simulink subsystem "PvtSubSys_VSM_ALL"  (R2020b)
settings: Solver=VariableStepAuto  StartTime=0.0  StopTime=10.0  RelTol=1e-3
values from neighbouring files (symbols this model uses):
  P_VSM_NOH_Act_Req = 0    [VSM_All.sldd]
  P_VSM_NOH_Swt_Req = 0    [VSM_All.sldd]
undefined symbols (not defined in the file or in its folder): ACC_STATE, HWA_STATE, LCK_STATE, P_VSM_ACCSOS_SW, P_VSM_AESSwtReq, P_VSM_CruiseFunUserInputMappingWays, P_VSM_ELKSwtReq, P_VSM_ESS_VehSwtReq, P_VSM_HWA_DMS_Enable, P_VSM_ICA_HandsOffSwtReq, P_VSM_IntelligentEvaSwtReq, P_VSM_ISLSwtReq, P_VSM_LCKSwtReq, P_VSM_LDWSwtReq, P_VSM_LKASwtReq, P_VSM_LSSSwtReq, P_VSM_PowerTrainConfig, P_VSM_SOSContinueTime, P_VSM_SOSSpdLimit, P_VSM_TSR_Dis_keep_SPL_Table, P_VSM_TSR_Dis_keep_SPLend, P_VSM_TSR_Dis_keep_TS_Table, P_VSM_TSR_Ena_SPLSupp_Table, P_VSM_TSR_Ena_TS_Table, P_VSM_TSR_SLIF_Speed_High, P_VSM_TSR_SLIF_Speed_Low, P_VSM_TSR_SLW_SnvtySwitch, P_VSM_TSR_SLW_Speed_Delta_disable, P_VSM_TSR_SLW_Speed_Delta_enable, P_VSM_TSR_SLW_Speed_High, P_VSM_TSR_SLW_Speed_Low, P_VSM_TSR_SLW_TrafEyeAvtiveDist, P_VSM_TSR_SLW_Warning_Time, P_VSM_TSR_SteerWheelAngle, P_VSM_TSR_SWS_speed_withDir, P_VSM_TSR_SWS_speed_woDir, P_VSM_TSRSwtReq, P_VSM_TSRWarnSwtReq, TJA_STATE, User_LC_ALCswt, User_LC_DrvConfirm, User_LC_DrvLCswt, User_LC_DrvOverride, User_LC_LeTurnNextLineReq, User_LC_RiTurnNextLineReq, User_LC_TurnMostLeLineReq, User_LC_TurnMostRiLineReq, User_LeTurnLmpOn, User_RiTurnLmpOn
libraries: simulink x51
(part 2 of 7)

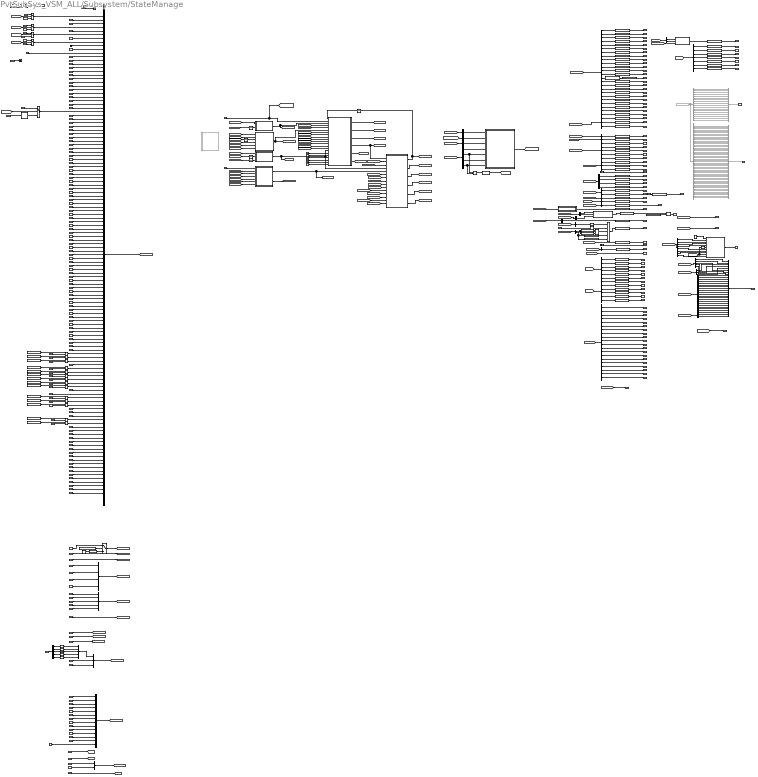
== system PvtSubSys_VSM_ALL/Subsystem/StateManage ==
  note: GotoFrom颜色说明
      | 前景色-背景色
      | Black-Orange 模块输入(连接到本模块输入端口)
      | Black-Cyan 模块输出(仅连接到本模块输出端口)
      | Blue-Cyan 模块输出(连接到本模块输出端口同时被其他模块使用)
      | Blue-others 内部跳转(未连接到本模块输入输入端口)
      | Black-White 未指定/其他
  note: 0:ICE
      | 1:PHEV
  note: 版本管理
      | VSM
      | 20201203-4.0
      | 初版
  note: 换道点灯信号
  note: 配置自
  note: 诊断
  note: 脱手检测
  EngState_PHEV : Inport  OutDataTypeStr=uint8  PortDimensions=1
  EngSpd : Inport  Port=2  OutDataTypeStr=single  PortDimensions=1
  EngState : Inport  Port=3
  BrkPedalSts : Inport  Port=4
  Start_StopSts : Inport  Port=5
  AccPedalOverride : Inport  Port=6
  AccelPedlPosnDiagc : Inport  Port=7
  ECMRespACC : Inport  Port=8
  ECMACCInterface : Inport  Port=9
  AccelPedalPosn : Inport  Port=10
  EngLimpHomeSts : Inport  Port=11
  CurrentGearValid : Inport  Port=12  OutDataTypeStr=boolean  PortDimensions=1
  SHIFT_IN_PROGRESS : Inport  Port=13  OutDataTypeStr=boolean  PortDimensions=1
  TargetGearValid : Inport  Port=14  OutDataTypeStr=boolean  PortDimensions=1
  TARGET_GEAR : Inport  Port=15  OutDataTypeStr=uint8  PortDimensions=1
  ShiftInPrgValid : Inport  Port=16  OutDataTypeStr=boolean  PortDimensions=1
  CURRENT_GEAR : Inport  Port=17  OutDataTypeStr=uint8  PortDimensions=1
  TGS_LEVER : Inport  Port=18  OutDataTypeStr=uint8  PortDimensions=1
  HCU_BrkPedalSts : Inport  Port=19  OutDataTypeStr=uint8  PortDimensions=1
  HCU_AccelPedalPosn_Diag : Inport  Port=20  OutDataTypeStr=single  PortDimensions=1
  HCU_ACCInterface : Inport  Port=21  OutDataTypeStr=boolean  PortDimensions=1
  HCU_PowertrainSts : Inport  Port=22  OutDataTypeStr=uint8  PortDimensions=1
  ACU_ShiftInProgress : Inport  Port=23  OutDataTypeStr=boolean  PortDimensions=1
  HCU_DrvMod : Inport  Port=24  OutDataTypeStr=uint8  PortDimensions=1
  HCU_PTDrvMod : Inport  Port=25  OutDataTypeStr=uint8  PortDimensions=1
  DrvTrqReqOvld : Inport  Port=26  OutDataTypeStr=boolean  PortDimensions=1
  HCU_GearSts : Inport  Port=27  OutDataTypeStr=uint8  PortDimensions=1
  DrivingModDis : Inport  Port=28
  BrkDskOvrheatd : Inport  Port=29  OutDataTypeStr=boolean  PortDimensions=1
  NoBrkForce : Inport  Port=30  OutDataTypeStr=boolean  PortDimensions=1
  VehStandstill : Inport  Port=31  OutDataTypeStr=uint8  PortDimensions=1
  HDCCtrl : Inport  Port=32  OutDataTypeStr=uint8  PortDimensions=1
  CDDActv : Inport  Port=33  OutDataTypeStr=boolean  PortDimensions=1
  CDDAvailable : Inport  Port=34  OutDataTypeStr=boolean  PortDimensions=1
  AVHSts : Inport  Port=35  OutDataTypeStr=uint8  PortDimensions=1
  ESPFuncOffSts : Inport  Port=36  OutDataTypeStr=boolean  PortDimensions=1
  ESPBrkLmpCtrl : Inport  Port=37  OutDataTypeStr=boolean  PortDimensions=1
  ESPFailSts : Inport  Port=38  OutDataTypeStr=boolean  PortDimensions=1
  ESP_MasterCylBrkPressVld : Inport  Port=39  OutDataTypeStr=boolean  PortDimensions=1
  MSRActv : Inport  Port=40  OutDataTypeStr=boolean  PortDimensions=1
  VDCActv : Inport  Port=41  OutDataTypeStr=boolean  PortDimensions=1
  PTCActv : Inport  Port=42  OutDataTypeStr=boolean  PortDimensions=1
  BTCActv : Inport  Port=43  OutDataTypeStr=boolean  PortDimensions=1
  ESP_MasterCylBrkPress : Inport  Port=44  OutDataTypeStr=single  PortDimensions=1
  MSRActv_RA : Inport  Port=45  OutDataTypeStr=boolean  PortDimensions=1
  PTCActv_RA : Inport  Port=46  OutDataTypeStr=boolean  PortDimensions=1
  BTCActv_RA : Inport  Port=47  OutDataTypeStr=boolean  PortDimensions=1
  ABSFailSts : Inport  Port=48  OutDataTypeStr=boolean  PortDimensions=1
  EBDFailSts : Inport  Port=49  OutDataTypeStr=boolean  PortDimensions=1
  VehSpd : Inport  Port=50  OutDataTypeStr=single  PortDimensions=1
  ABSActv : Inport  Port=51  OutDataTypeStr=boolean  PortDimensions=1
  EPBSts : Inport  Port=52  OutDataTypeStr=uint8  PortDimensions=1
  EPB_SwtPosn : Inport  Port=53  OutDataTypeStr=uint8  PortDimensions=1
  RLWheelDriveDirection : Inport  Port=54  OutDataTypeStr=uint8  PortDimensions=1
  RLWheelSpd : Inport  Port=55  OutDataTypeStr=single  PortDimensions=1
  RRWheelDriveDirection : Inport  Port=56  OutDataTypeStr=uint8  PortDimensions=1
  RRWheelSpd : Inport  Port=57  OutDataTypeStr=single  PortDimensions=1
  EPS_FailSts : Inport  Port=58  OutDataTypeStr=uint8  PortDimensions=1
  EPS_TrqSnsrSts : Inport  Port=59  OutDataTypeStr=boolean  PortDimensions=1
  EPS_SteerMod : Inport  Port=60  OutDataTypeStr=uint8  PortDimensions=1
  EPS_LKATorqOvrlDlvd : Inport  Port=61  OutDataTypeStr=single  PortDimensions=1
  EPS_LKATorqOvrlDlvdVld : Inport  Port=62  OutDataTypeStr=boolean  PortDimensions=1
  EPS_LKATrqOvlDlvdSts : Inport  Port=63  OutDataTypeStr=uint8  PortDimensions=1
  EPS_DrvInpTrqVal_HighReslolution : Inport  Port=64  OutDataTypeStr=single  PortDimensions=1
  SysPowerMod : Inport  Port=65  OutDataTypeStr=uint8  PortDimensions=1
  WiprReq : Inport  Port=66  OutDataTypeStr=uint8  PortDimensions=1
  DrvDoorSts : Inport  Port=67  OutDataTypeStr=boolean  PortDimensions=1
  PassengerDoorSts : Inport  Port=68  OutDataTypeStr=boolean  PortDimensions=1
  WindshldWiprActvSts : Inport  Port=69  OutDataTypeStr=boolean  PortDimensions=1
  HazardLmpSwtSts : Inport  Port=70  OutDataTypeStr=boolean  PortDimensions=1
  "KL30BRelaySts " : Inport  Port=71  OutDataTypeStr=boolean  PortDimensions=1
  ACAmbTemp : Inport  Port=72  OutDataTypeStr=single  PortDimensions=1
  HoodSts_F_Pbox : Inport  Port=73  OutDataTypeStr=boolean  PortDimensions=1
  FFogLmpSts_F_Pbox : Inport  Port=74  OutDataTypeStr=boolean  PortDimensions=1
  RFogLmpSts_R_Pbox : Inport  Port=75  OutDataTypeStr=boolean  PortDimensions=1
  LowBeamSts : Inport  Port=76  OutDataTypeStr=boolean  PortDimensions=1
  FrntWshrSwtSts : Inport  Port=77  OutDataTypeStr=uint8  PortDimensions=1
  FrntWiprSwtSts : Inport  Port=78  OutDataTypeStr=uint8  PortDimensions=1
  LTurnLmpSwtSts : Inport  Port=79  OutDataTypeStr=boolean  PortDimensions=1
  RTurnLmpSwtSts : Inport  Port=80  OutDataTypeStr=boolean  PortDimensions=1
  SteerWheelAng : Inport  Port=81  OutDataTypeStr=single  PortDimensions=1
  SteerWheelAngSign : Inport  Port=82  OutDataTypeStr=boolean  PortDimensions=1
  SteerWheelSpd : Inport  Port=83  OutDataTypeStr=single  PortDimensions=1
  SteerWheelSpdSign : Inport  Port=84  OutDataTypeStr=boolean  PortDimensions=1
  SAS_Sts : Inport  Port=85  OutDataTypeStr=uint8  PortDimensions=1
  ACC_TimeGap_IncSetSwt : Inport  Port=86  OutDataTypeStr=boolean  PortDimensions=1
  ACC_TimeGap_DecSetSwt : Inport  Port=87  OutDataTypeStr=boolean  PortDimensions=1
  CC_ACC_CRUISE_OFFSwt : Inport  Port=88  OutDataTypeStr=boolean  PortDimensions=1
  CC_ACC_CANCEL_OFFSwt : Inport  Port=89  OutDataTypeStr=boolean  PortDimensions=1
  CC_ACC_IncSetSpd_ResuSwt : Inport  Port=90  OutDataTypeStr=boolean  PortDimensions=1
  CC_ACC_DecSetSpd_SetSwt : Inport  Port=91  OutDataTypeStr=boolean  PortDimensions=1
  CC_ACCSwtErr : Inport  Port=92  OutDataTypeStr=boolean  PortDimensions=1
  HWA_OK_OFFSwt : Inport  Port=93  OutDataTypeStr=boolean  PortDimensions=1
  DrvSBR : Inport  Port=94  OutDataTypeStr=boolean  PortDimensions=1
  PassSBR : Inport  Port=95  OutDataTypeStr=boolean  PortDimensions=1
  VehLgtAccel : Inport  Port=96  OutDataTypeStr=single  PortDimensions=1
  VehLatAccel : Inport  Port=97  OutDataTypeStr=single  PortDimensions=1
  VehYawRate : Inport  Port=98  OutDataTypeStr=single  PortDimensions=1
  IP_VehSpdUnit : Inport  Port=99  OutDataTypeStr=boolean  PortDimensions=1
  IFC_SnvtySet : Inport  Port=100  OutDataTypeStr=uint8  PortDimensions=1
  LKASwtReq : Inport  Port=101  OutDataTypeStr=boolean  PortDimensions=1
  LCKSwtReq : Inport  Port=102  OutDataTypeStr=boolean  PortDimensions=1
  ELKSwtReq : Inport  Port=103  OutDataTypeStr=boolean  PortDimensions=1
  ESS_PedSwtReq : Inport  Port=104  OutDataTypeStr=boolean  PortDimensions=1
  ESS_VehSwtReq : Inport  Port=105  OutDataTypeStr=boolean  PortDimensions=1
  LDWSwtReq : Inport  Port=106  OutDataTypeStr=boolean  PortDimensions=1
  TSRSwtReq : Inport  Port=107  OutDataTypeStr=boolean  PortDimensions=1
  TSRWarnSwtReq : Inport  Port=108  OutDataTypeStr=boolean  PortDimensions=1
  ICA_HandsOffSwtReq : Inport  Port=109  OutDataTypeStr=boolean  PortDimensions=1
  ISLSwtReq : Inport  Port=110  OutDataTypeStr=boolean  PortDimensions=1
  TSR_SnvtySet : Inport  Port=111  OutDataTypeStr=int8  PortDimensions=1
  LSSWarnFormSwtReq : Inport  Port=112  OutDataTypeStr=uint8  PortDimensions=1
  LSSSwtReq : Inport  Port=113  OutDataTypeStr=boolean  PortDimensions=1
  IntelligentEvaSwtReq : Inport  Port=114  OutDataTypeStr=boolean  PortDimensions=1
  AESSwtReq : Inport  Port=115  OutDataTypeStr=boolean  PortDimensions=1
  HWA_SwtReq : Inport  Port=116  OutDataTypeStr=boolean  PortDimensions=1
  HWA_SnvtySet : Inport  Port=117  OutDataTypeStr=uint8  PortDimensions=1
  ALC_SwtReq : Inport  Port=118  OutDataTypeStr=boolean  PortDimensions=1
  NOH_Act_Req : Inport  Port=119
  NOH_Swt_Req : Inport  Port=120
  NavRoadType : Inport  Port=121
  CR_BrkgReq : Inport  Port=122  OutDataTypeStr=boolean  PortDimensions=1
  HighBeamSts : Inport  Port=123  OutDataTypeStr=boolean  PortDimensions=1
  USS_FrontSys_Status : Inport  Port=124  OutDataTypeStr=uint8  PortDimensions=1
  USS_FLCNear_Obj_Confidence : Inport  Port=125  OutDataTypeStr=single  PortDimensions=1
  USS_FLCNear_Obj_Pos_X : Inport  Port=126  OutDataTypeStr=single  PortDimensions=1
  USS_FLCNear_Obj_Pos_Y : Inport  Port=127  OutDataTypeStr=single  PortDimensions=1
  USS_FLMNear_Obj_Confidence : Inport  Port=128  OutDataTypeStr=single  PortDimensions=1
  USS_FLMNear_Obj_Pos_X : Inport  Port=129  OutDataTypeStr=single  PortDimensions=1
  USS_FLMNear_Obj_Pos_Y : Inport  Port=130  OutDataTypeStr=single  PortDimensions=1
  USS_FRMNear_Obj_Confidence : Inport  Port=131  OutDataTypeStr=single  PortDimensions=1
  USS_FRMNear_Obj_Pos_X : Inport  Port=132  OutDataTypeStr=single  PortDimensions=1
  USS_FRMNear_Obj_Pos_Y : Inport  Port=133  OutDataTypeStr=single  PortDimensions=1
  USS_FRCNear_Obj_Confidence : Inport  Port=134  OutDataTypeStr=single  PortDimensions=1
  USS_FRCNear_Obj_Pos_X : Inport  Port=135  OutDataTypeStr=single  PortDimensions=1
  USS_FRCNear_Obj_Pos_Y : Inport  Port=136  OutDataTypeStr=single  PortDimensions=1
  APS_WorkSts : Inport  Port=137  OutDataTypeStr=uint8  PortDimensions=1
  DVRWorkSts : Inport  Port=138  OutDataTypeStr=uint8  PortDimensions=1
  DriverSts : Inport  Port=139  OutDataTypeStr=uint8  PortDimensions=1
  CAL_VSM_CONFIG : Inport  Port=140  OutDataTypeStr=Bus: CAL_VSM_CONFIG_BUS  PortDimensions=1
  DFIM_VSM_STS : Inport  Port=141  OutDataTypeStr=Bus: DFIM_VSM_STS_BUS  PortDimensions=1
  RFM_LINE_L1 : Inport  Port=142  OutDataTypeStr=Bus: RFM_LINE_BUS  PortDimensions=1
  RFM_LINE_R1 : Inport  Port=143  OutDataTypeStr=Bus: RFM_LINE_BUS  PortDimensions=1
  RFM_LINEF_LB : Inport  Port=144  OutDataTypeStr=Bus: RFM_LINE_BUS  PortDimensions=1
  RFM_LINEF_RB : Inport  Port=145  OutDataTypeStr=Bus: RFM_LINE_BUS  PortDimensions=1
  LSM_Cnt : Inport  Port=146  OutDataTypeStr=uint32  PortDimensions=1
  LSM_TJA_ICA : Inport  Port=147  OutDataTypeStr=Bus: LSM_TJA_ICA_BUS  PortDimensions=1
  LSM_HWA : Inport  Port=148  OutDataTypeStr=Bus: LSM_HWA_BUS  PortDimensions=1
  LSM_LCK : Inport  Port=149  OutDataTypeStr=Bus: LSM_LCK_BUS  PortDimensions=1
  LSM_ESS : Inport  Port=150  OutDataTypeStr=Bus: LSM_ESS_BUS  PortDimensions=1
  TOS_ACCP0 : Inport  Port=151  OutDataTypeStr=Bus: TOS_ACCP0_BUS  PortDimensions=1
  TOS_AEB_LONOBJ_BUS : Inport  Port=152  OutDataTypeStr=Bus: TOS_AEB_LONOBJ_BUS
  TOS_ELK : Inport  Port=153  OutDataTypeStr=Bus: TOS_ELK_BUS  PortDimensions=8
  TOS_LCKIE : Inport  Port=154  OutDataTypeStr=Bus: TOS_LCKIE_BUS  PortDimensions=9
  EHRV2_ALL : Inport  Port=155  Interpolate=off  BusOutputAsStruct=on
  IFCHUTInterface : Inport  Port=156  OutDataTypeStr=uint8  PortDimensions=1
  MapDataValid : Inport  Port=157  OutDataTypeStr=uint8  PortDimensions=1
  axvRefMs2 : Inport  Port=158  OutDataTypeStr=single  PortDimensions=1
  vxvRefMs : Inport  Port=159  OutDataTypeStr=single  PortDimensions=1
  axvRoadSlopeMs2 : Inport  Port=160  OutDataTypeStr=single  PortDimensions=1
  psiDtOpt : Inport  Port=161  OutDataTypeStr=single  PortDimensions=1
  ayvRefMs2 : Inport  Port=162  OutDataTypeStr=single  PortDimensions=1
  kapTraj : Inport  Port=163  OutDataTypeStr=single  PortDimensions=1
  AEB_VehResp : Inport  Port=164  OutDataTypeStr=boolean  PortDimensions=1
  AEB_PedResp : Inport  Port=165  OutDataTypeStr=boolean  PortDimensions=1
  Inter_FCW_Warn : Inport  Port=166  OutDataTypeStr=uint8  PortDimensions=1
  AEB_VehTrig : Inport  Port=167  OutDataTypeStr=boolean  PortDimensions=1
  AEB_PedTrig : Inport  Port=168  OutDataTypeStr=boolean  PortDimensions=1
  " " : Inport  Port=169  OutDataTypeStr=boolean  PortDimensions=1
  DriveOffConditionFulfilled : Inport  Port=170  OutDataTypeStr=boolean  PortDimensions=1
  RFM_TSR : Inport  Port=171  OutDataTypeStr=Bus: RFM_TSR_BUS  PortDimensions=1
  epsTrqReqValue : Inport  Port=172  OutDataTypeStr=single  PortDimensions=1
  epsTrqReqFlag : Inport  Port=173  OutDataTypeStr=uint8  PortDimensions=1
  VSM_TSR_INIT : Inport  Port=174  OutDataTypeStr=Bus: VSM_TSR_INIT_BUS  PortDimensions=1
  Longctrl_Decel_ReqValue : Inport  Port=175
  ALC : Inport  Port=176  OutDataTypeStr=Bus: PLAN_ALC_DECS_BUS  LockScale=on
  PLAN_DPC_ESS : Inport  Port=177  OutDataTypeStr=Bus: PLAN_DPC_ESS_BUS
  PilotSts : Inport  Port=178  OutDataTypeStr=uint8
  LSM_PilotNohExitDist : Inport  Port=179
  PLAN_NOH_SetSpdAdjReq : Inport  Port=180
  PLAN_NOH_SetSpdAdjVal : Inport  Port=181
  LSM_TJALineSource : Inport  Port=182
  TimeGapInit : Inport  Port=183
  IB_BrkPedalAppld : Inport  Port=184
  ConfigiBooster : Inport  Port=185
  AND : Logic  AllPortsSameDT=off  OutDataTypeStr=boolean
  Bus Assignment : BusAssignment  AssignedSignals=User_LeTurnLmpOn,User_RiTurnLmpOn,User_LC_LeTurnNextLineReq,User_LC_RiTurnNextLineReq,User_LC_TurnMostLeLineReq,User_LC_TurnMostRiLineReq,User_LC_ALCswt,User_LC_DrvConfirm,User_LC_DrvOverride,User_LC_DrvLCswt
  Bus Creator : BusCreator  Inputs=5
  Bus Creator1 : BusCreator  Inputs=3
  Bus Creator12 : BusCreator  Inputs=2
  Bus Creator19 : BusCreator  Inputs=14
  Bus Creator2 : BusCreator  Inputs=31
  Bus Creator3 : BusCreator  Inputs=131
  Bus Creator4 : BusCreator  Inputs=4
  Bus Creator5 : BusCreator  Inputs=5
  Bus Creator7 : BusCreator  Commented=on  Inputs=18  OutDataTypeStr=Bus: ACCExitConds  NonVirtualBus=on
  Bus Creator8 : BusCreator  Commented=on  Inputs=53  OutDataTypeStr=Bus: HWAExitConds  NonVirtualBus=on
  Bus Selector : BusSelector  OutputSignals=LCK_Con_SteerAngleSpd_ LCKExit,LCK_Con_OverRide_ LCKExit,LCK_Con_SteerWheelAngle_ LCKExit,LCK_Con_DriverInput_ LCKExit
  Bus Selector1 : BusSelector  OutputSignals=Signal_HandsOffWarn
  Bus Selector10 : BusSelector  OutputSignals=TSRSts,TSRResp,TSRWarnResp,TSR_Snvty,TSRSpdLimUnit,TSRSpdLimSts,TSRSpdLim,TSRSpdLimCfdc,TSRSpdLimWarn,TSRConSpdLim,TSRConSpdLimWarn,TSRTrfcSignVal,TSRTrfcSignValCfdc,SPL_noSupp_Dist_Remain,SPL_whSupp_Dist_Remain,TS_SignName_Dist_Remain,SPL_noSupp_Value_Remain,SPL_whSupp_Value_Remain,TS_SignName_Value_Remain,SPL_SuppName_Value_Remain
  Bus Selector11 : BusSelector  OutputSignals=LDW_Con_AccPedalRate_LDWExit,LDW_Con_BrakePressure_ LDWExit,LDW_Con_SteerWheelAngle_ LDWExit,LDW_Con_DriverInput_ LDWExit,LDW_Con_SteerWheelSpd_ LDWExit,LKA_Con_AccPedalRate_LKAExit,LKA_Con_BrakePressure_ LKAExit,LKA_Con_SteerWheelAngle_ LKAExit,LKA_Con_DriverInput_ LKAExit,LKA_Con_SteerWheelSpd_ LKAExit,LKA_Con_OverRide_ LKAExit,ELK_Con_AccPedalRate_ELKExit,ELK_Con_BrakePressure_ ELKExit,ELK_Con_SteerWheelAngle_ ELKExit,ELK_Con_SteerWheelSpd_ ELKExit,LCK_Con_AccPedalRate_LCKExit,LCK_Con_BrakePress_ LCKExit,LCK_Con_SteerAngleSpd_ LCKExit,LCK_Con_OverRide_ LCKExit,LCK_Con_SteerWheelAngle_ LCKExit,LCK_Con_DriverInput_ LCKExit
  Bus Selector12 : BusSelector  OutputSignals=LSM_TJA_ICA.TJALineValid
  Bus Selector13 : BusSelector  OutputSignals=HandsOffDetd
  Bus Selector14 : BusSelector  OutputSignals=i_func_road_class,i_form_of_way,f_tunnel_distance,f_start_distance,i_road_curvature_far
  Bus Selector15 : BusSelector  OutputSignals=ESSDataClct_OverrideESSExit,ESSDataClct_DriverSteerESSExit
  Bus Selector16 : BusSelector  OutputSignals=TJASts,VSM_HWASts
  Bus Selector17 : BusSelector  OutputSignals=NOH_Swt_Resp,NOH_Act_Resp,HiPilotModeSelect
  Bus Selector18 : BusSelector  OutputSignals=VSM_HWA_ParkShiftReq,TJASts
  Bus Selector19 : BusSelector  OutputSignals=Signal_ACC_ModeSts,Signal_ACC_SpdSetValue,Signal_ACC_TimeGapSet,vSetBelowMin,Signal_ACC_DrvOFF_Req,TJASts,VSM_HWASts,VSM_HWAActive,Signal_ACC_HazActv,Signal_ACC_ModDisp,Signal_ACC_ParkShiftReq,Signal_TJA_ModeSts,Signal_HWAModeDisp,VSM_HWASts,Signal_CruiseChauffer_Sts,Signal_ACCTextDisp,Signal_TJATextDisp,Signal_CCTextDisp,SetSpeedKmH,Signal_HWATextDisp,ACC_DrvrOffDisp,VSM_NOH_Sts,VSM_NOH_SysInfoDisplay,VSM_NOH_DistToExit
  Bus Selector2 : BusSelector  OutputSignals=LCK_State
  Bus Selector20 : BusSelector  OutputSignals=ISL_Resp,ISL_InterSysInfoDisp,ISL_Active
  Bus Selector21 : BusSelector  OutputSignals=ACCDataClct_OverrideACCExit
  Bus Selector22 : BusSelector  OutputSignals=VSM_TarLineValid,VSM_TarLineC3,VSM_TarLineC2,VSM_TarLineC1,VSM_TarLineC0,VSM_TarLineRange,VSM_TarDangerLevel
  Bus Selector23 : BusSelector  OutputSignals=VSM_HWAWarningLevel
  Bus Selector24 : BusSelector  OutputSignals=TJA_ACC_SelSts,VSM_HWA_LaneChangeReq
  Bus Selector25 : BusSelector  OutputSignals=VehSpd
  Bus Selector3 : BusSelector  OutputSignals=EDR_DriverBrakeHWAExit
  Bus Selector4 : BusSelector  OutputSignals=LCKIE_State
  Bus Selector43 : BusSelector  OutputSignals=VSM_LKALaneValid,VSM_LKALaneA3,VSM_LKALaneA2,VSM_LKALaneA1,VSM_LKALaneA0,VSM_LKALaneRange
  Bus Selector46 : BusSelector  OutputSignals=VSM_ELKLaneValid,VSM_ELKLaneA3,VSM_ELKLaneA2,VSM_ELKLaneA1,VSM_ELKLaneA0,VSM_ELKLaneRange
  Bus Selector47 : BusSelector  OutputSignals=LDW_State,LKA_State,LKAWarning,ELK_State,LCKIE_Laneoffset
  Bus Selector5 : BusSelector  OutputSignals=LTurnLmpSwtSts,RTurnLmpSwtSts,User_LC_LeTurnNextLineReq,User_LC_RiTurnNextLineReq,User_LC_TurnMostRiLineReq,User_LC_ALCswt,User_LC_DrvConfirm,User_LC_DrvLCswt
  Bus Selector57 : BusSelector  OutputSignals=ALC_SwtReq,HWA_SnvtySet,HWA_SwtReq,ICA_HandsOffSwtReq
  Bus Selector6 : BusSelector  OutputSignals=VSM_HWAActive
  Bus Selector60 : BusSelector  OutputSignals=LSSWarnFormSwtReq
  Bus Selector63 : BusSelector  OutputSignals=VSM_HWASts,TJASts
  Bus Selector7 : BusSelector  OutputSignals=LaneAvaliability
  Bus Selector75 : BusSelector  Commented=on  OutputSignals=ACCFastExit.VSM_ACCFastExitCons_Standstill3min,ACCFastExit.VSM_ACCFastExitCons_StandstillNoBrakeForce,ACCFastExit.VSM_ACCFastExitCons_RollingBack,ACCFastExit.VSM_ACCFastExitCons_EngineOff,ACCFastExit.VSM_ACCFastExitCons_BrakeDiskOverHeat,ACCFastExit.VSM_ACCFastExitCons_Cancel,ACCFastExit.VSM_ACCFastExitCons_EspOff,ACCFastExit.VSM_ACCFastExitCons_NoForwardGear,ACCFastExit.VSM_ACCFastExitCons_DriveBrakeExit,ACCFastExit.VSM_ACCFastExitCons_EPBClosed,ACCFastExit.VSM_ACCFastExitCons_DriverDoorOpen,ACCSlowExit.VSM_ACCSlowExitCons_EspActive400ms,ACCSlowExit.VSM_ACCSlowExitCons_MSRactive800ms,ACCSlowExit.VSM_ACCSlowExitCons_HDCactive40ms,ACCSlowExit.VSM_ACCSlowExitCons_ABSactive400ms,ACCSlowExit.VSM_ACCSlowExitCons_TCS1active3000ms,ACCSlowExit.VSM_ACCSlowExitCons_TCS2active3000ms,ACCSlowExit.VSM_ACCFastExitCons_DriverSBR
  Bus Selector76 : BusSelector  Commented=on  OutputSignals=HWASlowExitConditions.VSM_HWASlowExitCons_AEBTrigger,HWASlowExitConditions.VSM_HWASlowExitCons_AEBOff,HWASlowExitConditions.VSM_HWASlowExitCons_HandsoffOverride,HWASlowExitConditions.VSM_HWASlowExitCons_HighSpdIn3s,HWASlowExitConditions.VSM_HWASlowExitCons_DMSInvalid,HWASlowExitConditions.VSM_HWASlowExitCons_MapDataInvalid,HWASlowExitConditions.VSM_HWASlowExitCons_DVRError,HWASlowExitConditions.VSM_HWASlowExitCons_SingleLineLost,ACCSlowExit.VSM_ACCSlowExitCons_EspActive400ms,ACCSlowExit.VSM_ACCSlowExitCons_MSRactive800ms,ACCSlowExit.VSM_ACCSlowExitCons_HDCactive40ms,ACCSlowExit.VSM_ACCSlowExitCons_ABSactive400ms,ACCSlowExit.VSM_ACCSlowExitCons_TCS1active3000ms,ACCSlowExit.VSM_ACCSlowExitCons_TCS2active3000ms,ACCSlowExit.VSM_ACCFastExitCons_DriverSBR,HWASlowExitConditions.VSM_HWASlowExitCons_NotHighWayArterialRoad5s,HWASlowExitConditions.VSM_HWASlowExitCons_LCKIdleWithoutTurnLight,HWASlowExitConditions.VSM_HWASlowExitCons_HWAError_Inhibit,HWASlowExitConditions.VSM_HWASlowExitCons_HWAError_Error,HWASlowExitConditions.VSM_HWASlowExitCons_HWAError_ErrorBlindness,SomeHWASafeStop2ExitConds.VSM_HWAFastExitCons_ACCNotActive,SomeHWASafeStop2ExitConds.VSM_HWAFastExitCons_HWAErrorFastExit,SomeHWASafeStop2ExitConds.VSM_HWAFastExitCons_ParkGearOrEPBActive,SomeHWASafeStop2ExitConds.VSM_HWAFastExitCons_StandstillTimeout,SomeHWASafeStop2ExitConds.VSM_HWAFastExitCons_OverrideTimeout,SomeHWASafeStop2ExitConds.VSM_HWAFastExitCons_SpeedTooHighWithOverride,HWAActivationConds.VSM_HWAActivationCons_VehicleSpdNormal3s,HWAActivationConds.VSM_HWAActivationCons_TJAActive,HWAActivationConds.VSM_HWAActivationCons_LCKActive,HWAActivationConds.VSM_HWAActivationCons_HandsOn5s,HWAActivationConds.VSM_HWAActivationCons_DriverStsGood10s,HWAActivationConds.VSM_HWAActivationCons_AEBSwitchOn,HWAActivationConds.VSM_HWAActivationCons_HWALineValid,HWAActivationConds.VSM_HWAActivationCons_NoSingleLineLost,HWAActivationConds.VSM_HWAActivationCons_NoDoubleLineLost,HWAActivationConds.VSM_HWAActivationCons_HighWayArterialRoad,HWAActivationConds.VSM_HWAActivationCons_NoTunnel300m,HWAActivationConds.VSM_HWAActivationCons_NoForkRoad300m,HWAActivationConds.VSM_HWAActivationCons_MapDataValid,HWAActivationConds.VSM_HWAActivationCons_DVRNoError,HWAActivationConds.VSM_HWAActivationCons_NoHWANoError,HWAActivationConds.VSM_HWAActivationCons_NoHWASafeStopHappened_b,HWAActivationConds.VSM_HWAActivationCons_NoHWAFastExitConditions_b,HWADriveOffConds.DoubleLineNotLostOrP0TargetExist,HWADriveOffConds.DrivingOnHighWay,HWADriveOffConds.FormOfWay,HWADriveOffConds.MapDataValid,HWADriveOffConds.HWANoError,HWADriveOffConds.LTurnLightSwOff,HWADriveOffConds.RTurnLightSwOff,HWADriveOffConds.HazardLmpSwtStsOff,HWADriveOffConds.DriverStsGood,HWADriveOffConds.AEBSwitchOn
  Bus Selector8 : BusSelector  OutputSignals=ACCDataClct_ConNotStsf,TJADataClct_ConNotStsf,ACCDataClct_OverrideACCExit,ACCDataClct_DriverBrakeACCExit,ACCDataClct_DriverSteerACCExit
  Bus Selector9 : BusSelector  OutputSignals=HWADATAClct_OverrideHWAExit,HWADATAClct_DriverBrakeHWAExit,HWADATAClct_DriverSteerHWAExit
  Compare To Constant : simulink/Logic and Bit Operations/Compare To Constant  relop===  const=0  OutDataTypeStr=boolean
  Compare To Constant1 : simulink/Logic and Bit Operations/Compare To Constant  relop===  const=1  OutDataTypeStr=boolean
  Compare To Constant2 : simulink/Logic and Bit Operations/Compare To Constant  relop===  const=1  OutDataTypeStr=boolean
  Compare To Constant3 : simulink/Logic and Bit Operations/Compare To Constant  relop=~=  const=HWA_STATE.HWA_LeftTurn  OutDataTypeStr=boolean
  Compare To Constant4 : simulink/Logic and Bit Operations/Compare To Constant  relop=~=  const=HWA_STATE.HWA_RightTurn  OutDataTypeStr=boolean
  Compare To Constant5 : simulink/Logic and Bit Operations/Compare To Constant  relop===  const=TJA_STATE.TJA_SafeStop  OutDataTypeStr=boolean
  Compare To Constant6 : simulink/Logic and Bit Operations/Compare To Constant  relop===  const=HWA_STATE.HWA_SlowRetreat  OutDataTypeStr=boolean
  Compare To Constant63 : simulink/Logic and Bit Operations/Compare To Constant  relop===  const=TJA_STATE.TJA_Active  OutDataTypeStr=boolean
  Compare To Constant7 : simulink/Logic and Bit Operations/Compare To Constant  relop===  const=TJA_STATE.TJA_SlowRetreat  OutDataTypeStr=boolean
  Compare To Zero : simulink/Logic and Bit Operations/Compare To Zero  relop=~=  OutDataTypeStr=boolean
  Constant : Constant  Value=P_VSM_LKASwtReq
  Constant1 : Constant  Value=P_VSM_NOH_Act_Req
  Constant10 : Constant  Value=P_VSM_ISLSwtReq
  Constant11 : Constant  Value=P_VSM_NOH_Swt_Req
  Constant12 : Constant  Value=P_VSM_LSSSwtReq
  Constant13 : Constant  Value=P_VSM_IntelligentEvaSwtReq
  Constant14 : Constant  Value=P_VSM_AESSwtReq
  Constant15 : Constant  Value=0  OutDataTypeStr=Bus: VSM_UOM_LC_BUS
  Constant16 : Constant  Value=P_VSM_HWA_DMS_Enable
  Constant17 : Constant
  Constant18 : Constant  Value=P_VSM_ACCSOS_SW
  Constant2 : Constant  Value=P_VSM_LCKSwtReq
  Constant3 : Constant  Value=P_VSM_ELKSwtReq
  Constant4 : Constant  Value=P_VSM_PowerTrainConfig
  Constant5 : Constant  Value=P_VSM_ESS_VehSwtReq
  Constant6 : Constant  Value=P_VSM_LDWSwtReq
  Constant7 : Constant  Value=P_VSM_TSRSwtReq
  Constant8 : Constant  Value=P_VSM_TSRWarnSwtReq
  Constant9 : Constant  Value=P_VSM_ICA_HandsOffSwtReq
  Cruise : Subsystem
  Data Type Conversion : DataTypeConversion
  Data Type Conversion1 : DataTypeConversion  OutDataTypeStr=uint8
  Direct Lookup Table (n-D) : LookupNDDirect  NumberOfTableDimensions=1  Table=[0 0 0 0 0 2 3 4 0 0]  TableDataTypeStr=uint8
  EDR_HWAExit : Subsystem
  ESS : Subsystem
  Enlong2s1 : Subsystem
  From16 : From  Commented=on  GotoTag=HWAStateInfo
  Ground5 : Ground
  HOD : Subsystem
  LSS : Subsystem
  Logical Operator : Logic  Inputs=5  AllPortsSameDT=off  OutDataTypeStr=boolean
  Logical Operator1 : Logic  Operator=OR  AllPortsSameDT=off  OutDataTypeStr=boolean
  Logical Operator2 : Logic  Operator=OR  Inputs=3  AllPortsSameDT=off  OutDataTypeStr=boolean
  MATLAB Function2 : MATLAB Function  TreatAsAtomicUnit=on
  MATLAB Function4 : MATLAB Function  TreatAsAtomicUnit=on
  OR{,1..9,12,14..15} (13 alike) : Logic  Operator=OR  AllPortsSameDT=off  OutDataTypeStr=boolean
  OR10 : Logic  Operator=OR  IconShape=distinctive  AllPortsSameDT=off  OutDataTypeStr=boolean
  Signal Copy{,1..4} (5 alike) : SignalConversion  OverrideOpt=off
  Switch{,1..3,5..6} (6 alike) : Switch  Criteria=u2 ~= 0
  TSR : Subsystem
  TSR2 : Subsystem  Commented=on
  Terminator : Terminator
  Terminator8 : Terminator
  Terminator9 : Terminator
  UOM : Subsystem
  Unit Delay{,1..4} (5 alike) : UnitDelay  SampleTime=-1  HasFrameUpgradeWarning=on
  tt1 : Ground
  tt8 : Ground
  tt9 : Ground
  w{1,3..14,32..42,106..108,110,115..119,157,289,304,315,371..372,430..454,459..466} (72 alike) : DataTypeConversion
  w2 : DataTypeConversion  OutDataTypeStr=single
  ACCSts : Outport  OutDataTypeStr=uint8  PortDimensions=1
  ACC_SpdSetValue : Outport  Port=2  OutDataTypeStr=uint8  PortDimensions=1
  SetSpeedKmh : Outport  Port=3  OutDataTypeStr=single
  ACC_TimeGapSet : Outport  Port=4  OutDataTypeStr=uint8  PortDimensions=1
  vSetBelowMin : Outport  Port=5  OutDataTypeStr=boolean  PortDimensions=1
  HWAAccControlSts : Outport  Port=6  OutDataTypeStr=uint8  PortDimensions=1
  ACC_DrvOffReq : Outport  Port=7  OutDataTypeStr=boolean  PortDimensions=1
  ACC_TimeGapSetHMI : Outport  Port=8
  TarLineValid : Outport  Port=9  OutDataTypeStr=boolean  PortDimensions=1
  TarLineC3 : Outport  Port=10  OutDataTypeStr=single  PortDimensions=1
  TarLineC2 : Outport  Port=11  OutDataTypeStr=single  PortDimensions=1
  TarLineC1 : Outport  Port=12  OutDataTypeStr=single  PortDimensions=1
  TarLineC0 : Outport  Port=13  OutDataTypeStr=single  PortDimensions=1
  TarLineRange : Outport  Port=14  OutDataTypeStr=single  PortDimensions=1
  TarDangerLevel : Outport  Port=15  OutDataTypeStr=uint8  PortDimensions=1
  TJASts : Outport  Port=16  OutDataTypeStr=uint8  PortDimensions=1
  HWASts : Outport  Port=17  OutDataTypeStr=uint8  PortDimensions=1
  HWAActive : Outport  Port=18  OutDataTypeStr=boolean  PortDimensions=1
  ACC_HazActv : Outport  Port=19  OutDataTypeStr=uint8  PortDimensions=1
  ACC_ModeDisp : Outport  Port=20  OutDataTypeStr=uint8  PortDimensions=1
  ACC_ParkShiftReq : Outport  Port=21  OutDataTypeStr=boolean  PortDimensions=1
  TJA_ModeDisp : Outport  Port=22  OutDataTypeStr=uint8  PortDimensions=1
  HWA_ModeDisp : Outport  Port=23  OutDataTypeStr=uint8  PortDimensions=1
  HWASlowRetreat_b : Outport  Port=24  OutDataTypeStr=boolean  PortDimensions=1
  CruiseChauffeur_ModeDisp : Outport  Port=25  OutDataTypeStr=uint8  PortDimensions=1
  ACCTextDisp : Outport  Port=26  OutDataTypeStr=uint8  PortDimensions=1
  TJATextDisp : Outport  Port=27  OutDataTypeStr=uint8  PortDimensions=1
  CCTextDisp : Outport  Port=28  OutDataTypeStr=uint8  PortDimensions=1
  HWATextDisp : Outport  Port=29  OutDataTypeStr=uint8  PortDimensions=1
  LCKSts : Outport  Port=30  OutDataTypeStr=uint8  PortDimensions=1
  HandsOffWarningLevel : Outport  Port=31  OutDataTypeStr=uint8  PortDimensions=1
  LDWSts : Outport  Port=32  OutDataTypeStr=uint8  PortDimensions=1
  LKASts : Outport  Port=33  OutDataTypeStr=uint8  PortDimensions=1
  LKAWarning : Outport  Port=34  OutDataTypeStr=uint8  PortDimensions=1
  ELKSts : Outport  Port=35  OutDataTypeStr=uint8  PortDimensions=1
  LCKIEDist : Outport  Port=36  OutDataTypeStr=single  PortDimensions=1
  ACC_ISLResp : Outport  Port=37  OutDataTypeStr=boolean  PortDimensions=1
  ISL_InterSysInfoDisp : Outport  Port=38  OutDataTypeStr=uint8  PortDimensions=1
  ISLActive : Outport  Port=39  OutDataTypeStr=uint8  PortDimensions=1
  EPBTakeOver_Req : Outport  Port=40  OutDataTypeStr=boolean  PortDimensions=1
  ALC_Resp : Outport  Port=41  OutDataTypeStr=boolean  PortDimensions=1
  HWA_SnvtySet_Resp : Outport  Port=42  OutDataTypeStr=uint8  PortDimensions=1
  HWA_Resp : Outport  Port=43  OutDataTypeStr=boolean  PortDimensions=1
  ICA_HandsOffSwtResp : Outport  Port=44  OutDataTypeStr=boolean  PortDimensions=1
  TJA_ACC_SelSts : Outport  Port=45  OutDataTypeStr=uint8  PortDimensions=1
  HWA_LaneChangeReq : Outport  Port=46  OutDataTypeStr=uint8  PortDimensions=1
  HWA_Warning : Outport  Port=47  OutDataTypeStr=uint8  PortDimensions=1
  HandsOffDetd : Outport  Port=48  OutDataTypeStr=boolean  PortDimensions=1
  LSS_WarnFormSwtResp : Outport  Port=49  OutDataTypeStr=uint8  PortDimensions=1
  DriverInloop_Monitor : Outport  Port=50  OutDataTypeStr=uint8  PortDimensions=1
  ACC_SOS_Req : Outport  Port=51  OutDataTypeStr=boolean  PortDimensions=1
  LaneAvailability : Outport  Port=52  OutDataTypeStr=uint8  PortDimensions=1
  TJA_FollowSts : Outport  Port=53  OutDataTypeStr=uint8  PortDimensions=1
  ESSSts : Outport  Port=54  OutDataTypeStr=uint8  PortDimensions=1
  AESSts : Outport  Port=55  OutDataTypeStr=uint8  PortDimensions=1
  LCKIESts : Outport  Port=56
  HWA_TurnLightReq : Outport  Port=57  OutDataTypeStr=uint8
  Signal_DriverOffDisp : Outport  Port=58  OutDataTypeStr=uint8  PortDimensions=1
  NOH_Sts : Outport  Port=59  OutDataTypeStr=uint8  PortDimensions=1
  NOH_Swt_Resp : Outport  Port=60  OutDataTypeStr=boolean  PortDimensions=1
  NOH_Act_Resp : Outport  Port=61  OutDataTypeStr=boolean  PortDimensions=1
  NOH_SysInfoDisplay : Outport  Port=62  OutDataTypeStr=uint8  PortDimensions=1
  NOH_DistToExit : Outport  Port=63  OutDataTypeStr=uint16  PortDimensions=1
  HiPilotModeSelect : Outport  Port=64  OutDataTypeStr=uint8  PortDimensions=1
  HWA_LaneChange : Outport  Port=65  OutDataTypeStr=uint8  PortDimensions=1
  LKALineValid : Outport  Port=66  OutDataTypeStr=boolean  PortDimensions=1
  LKALineC3 : Outport  Port=67  OutDataTypeStr=single  PortDimensions=1
  LKALineC2 : Outport  Port=68  OutDataTypeStr=single  PortDimensions=1
  LKALineC1 : Outport  Port=69  OutDataTypeStr=single  PortDimensions=1
  LKALineC0 : Outport  Port=70  OutDataTypeStr=single  PortDimensions=1
  LKALineRange : Outport  Port=71  OutDataTypeStr=single  PortDimensions=1
  ELKLineValid : Outport  Port=72  OutDataTypeStr=boolean  PortDimensions=1
  ELKLineC3 : Outport  Port=73  OutDataTypeStr=single  PortDimensions=1
  ELKLineC2 : Outport  Port=74  OutDataTypeStr=single  PortDimensions=1
  ELKLineC1 : Outport  Port=75  OutDataTypeStr=single  PortDimensions=1
  ELKLineC0 : Outport  Port=76  OutDataTypeStr=single  PortDimensions=1
  ELKLineRange : Outport  Port=77  OutDataTypeStr=single  PortDimensions=1
  TSRSts : Outport  Port=78  OutDataTypeStr=uint8  PortDimensions=1
  TSRResp : Outport  Port=79  OutDataTypeStr=boolean  PortDimensions=1
  TSRWarnResp : Outport  Port=80  OutDataTypeStr=boolean  PortDimensions=1
  TSR_Snvty : Outport  Port=81  OutDataTypeStr=int8  PortDimensions=1
  TSRSpdLimUnit : Outport  Port=82  OutDataTypeStr=uint8  PortDimensions=1
  TSRSpdLimSts : Outport  Port=83  OutDataTypeStr=uint8  PortDimensions=1
  TSRSpdLim : Outport  Port=84  OutDataTypeStr=uint8  PortDimensions=1
  TSRSpdLimCfdc : Outport  Port=85  OutDataTypeStr=uint8  PortDimensions=1
  TSRSpdLimWarn : Outport  Port=86  OutDataTypeStr=boolean  PortDimensions=1
  TSRConSpdLim : Outport  Port=87  OutDataTypeStr=uint8  PortDimensions=1
  TSRConSpdLimWarn : Outport  Port=88  OutDataTypeStr=boolean  PortDimensions=1
  TSRTrfcSignVal : Outport  Port=89  OutDataTypeStr=uint8  PortDimensions=1
  TSRTrfcSignValCfdc : Outport  Port=90  OutDataTypeStr=uint8  PortDimensions=1
  SPL_noSupp_Dist_Remain : Outport  Port=91  OutDataTypeStr=single  PortDimensions=1
  SPL_whSupp_Dist_Remain : Outport  Port=92  OutDataTypeStr=single  PortDimensions=1
  TS_SignName_Dist_Remain : Outport  Port=93  OutDataTypeStr=single  PortDimensions=1
  SPL_noSupp_Value_Remain : Outport  Port=94  OutDataTypeStr=uint8  PortDimensions=1
  SPL_whSupp_Value_Remain : Outport  Port=95  OutDataTypeStr=uint8  PortDimensions=1
  TS_SignName_Value_Remain : Outport  Port=96  OutDataTypeStr=uint8  PortDimensions=1
  SPL_SuppName_Value_Remain : Outport  Port=97  OutDataTypeStr=uint8  PortDimensions=1
  VSM_UOM_LC : Outport  Port=98
  DangerPlausMatrix : Outport  Port=99
  ACCExitConds : Outport  Port=100
  HWAExitConds : Outport  Port=101
  LSMC_Debug : Outport  Port=102
  LCK_Debugold : Outport  Port=103
  VSM_DATACLCT_INFO : Outport  Port=104
  wires:
  [ALC] -> LSS/15(ALC)
  Signal Copy4/1 -> Bus Creator5/5  "i_road_curvature_far"
  Bus Selector14/5 -> Signal Copy4/1  "<i_road_curvature_far>"
  ConfigiBooster/1 -> Cruise/21(ConfigiBooster)
  IB_BrkPedalAppld/1 -> Cruise/20(IB_BrkPedalAppld)
  Bus Selector25/1 -> Enlong2s1/3(vehspd)  "<VehSpd>"
  [AD_CAN] -> Bus Selector25/1
  Bus Selector18/2 -> Enlong2s1/2(TJASts)  "<TJASts>"
  TimeGapInit/1 -> Cruise/19(TimeGapInit)
  [ACC_TimeGapSetHMI] -> ACC_TimeGapSetHMI/1
  Cruise/6(ACC_TimeGapSetHMI) -> [ACC_TimeGapSetHMI]
  Compare To Zero/1 -> Bus Assignment/6
  [EDR_ACCDataClct] -> Bus Selector21/1
  Constant18/1 -> AND/2
  AND/1 -> ACC_SOS_Req/1
  Data Type Conversion1/1 -> [DirverOverride]
  LSM_TJALineSource/1 -> Compare To Constant2/1
  tt1/1 -> w14/1
  w14/1 -> HWA_LaneChange/1  "HWA_LaneChange"
  Bus Selector5/8 -> Bus Assignment/11  "<User_LC_DrvLCswt>"
  Compare To Constant7/1 -> Logical Operator2/3
  Bus Selector16/2 -> Compare To Constant3/1, Compare To Constant4/1  "<VSM_HWASts>"
  Compare To Constant5/1 -> Logical Operator2/2
  Compare To Constant63/1 -> Logical Operator2/1
  Compare To Constant4/1 -> Logical Operator/5
  Compare To Constant3/1 -> Logical Operator/4
  Switch6/1 -> [DriverSts]  "DriverSts"
  Constant17/1 -> Data Type Conversion/1
  Constant16/1 -> Switch6/2
  Data Type Conversion/1 -> Switch6/3
  Bus Selector5/7 -> Bus Assignment/9  "<User_LC_DrvConfirm>"
  Bus Selector5/6 -> Bus Assignment/8  "<User_LC_ALCswt>"
  Bus Selector5/5 -> Bus Assignment/7  "<User_LC_TurnMostRiLineReq>"
  Bus Selector5/4 -> Bus Assignment/5  "<User_LC_RiTurnNextLineReq>"
  Bus Selector5/3 -> Bus Assignment/4  "<User_LC_LeTurnNextLineReq>"
  Bus Selector5/1 -> Bus Assignment/2  "<LTurnLmpSwtSts>"
  Bus Selector5/2 -> Bus Assignment/3  "<RTurnLmpSwtSts>"
  Bus Assignment/1 -> VSM_UOM_LC/1
  Constant15/1 -> Bus Assignment/1
  OR10/1 -> Data Type Conversion1/1
  Enlong2s1/1(Out1) -> w12/1
  Bus Selector18/1 -> Enlong2s1/1(VSM_HWA_ParkShiftReq)  "<VSM_HWA_ParkShiftReq>"
  [HWAStateInfo] -> Bus Selector18/1
  Bus Selector19/18 -> w108/1  "<Signal_CCTextDisp>"
  Bus Selector17/3 -> w11/1  "<HiPilotModeSelect>"
  w11/1 -> HiPilotModeSelect/1  "HiPilotModeSelect"
  Bus Selector19/23 -> w9/1  "<VSM_NOH_SysInfoDisplay>"
  Bus Selector19/24 -> w10/1  "<VSM_NOH_DistToExit>"
  w10/1 -> NOH_DistToExit/1  "VSM_NOH_DistToExit"
  w9/1 -> NOH_SysInfoDisplay/1  "NOH_SysInfoDisplay"
  Bus Selector17/2 -> w8/1  "<NOH_Act_Resp>"
  w8/1 -> NOH_Act_Resp/1  "NOH_Act_Resp"
  w7/1 -> NOH_Swt_Resp/1  "NOH_Swt_Resp"
  Bus Selector17/1 -> w7/1  "<NOH_Swt_Resp>"
  [UserOperation] -> Bus Selector17/1
  Bus Selector19/22 -> w6/1  "<VSM_NOH_Sts>"
  w6/1 -> NOH_Sts/1  "NOH_Sts"
  LSM_PilotNohExitDist/1 -> Cruise/18(LSM_PilotNohExitDist)
  Bus Selector19/21 -> w5/1  "<ACC_DrvrOffDisp>"
  w5/1 -> Signal_DriverOffDisp/1  "ACC_DrvrOffDisp"
  Constant11/1 -> Logical Operator1/1
  Constant1/1 -> OR3/1
  NOH_Swt_Req/1 -> Logical Operator1/2  "NOH_Swt_Req"
  NOH_Act_Req/1 -> OR3/2  "NOH_Act_Req"
  NavRoadType/1 -> Bus Creator3/113  "NavRoadType"
  Logical Operator1/1 -> Bus Creator3/112  "NOH_Swt_Req"
  OR3/1 -> Bus Creator3/111  "NOH_Act_Req"
  Logical Operator2/1 -> Logical Operator/3
  Bus Selector16/1 -> Compare To Constant5/1, Compare To Constant7/1, Compare To Constant63/1  "<TJASts>"
  Compare To Constant2/1 -> Logical Operator/2
  Compare To Constant1/1 -> Logical Operator/1
  [HWAStateInfo] -> Bus Selector16/1
  Bus Selector12/1 -> Compare To Constant1/1  "<TJALineValid>"
  Logical Operator/1 -> w465/1
  [Target_Line] -> Bus Selector12/1
  Bus Selector11/12 -> Bus Creator2/20  "<ELK_Con_AccPedalRate_ELKExit>"
  Bus Selector11/8 -> Bus Creator2/16  "<LKA_Con_SteerWheelAngle_ LKAExit>"
  Bus Creator2/1 -> VSM_DATACLCT_INFO/1
  Bus Selector8/2 -> Bus Creator2/2  "<TJADataClct_ConNotStsf>"
  Bus Selector9/3 -> Bus Creator2/5  "<HWADATAClct_DriverSteerHWAExit>"
  Bus Selector11/6 -> Bus Creator2/14  "<LKA_Con_AccPedalRate_LKAExit>"
  [LSS_DATA] -> Bus Selector11/1
  Bus Selector11/14 -> Bus Creator2/22  "<ELK_Con_SteerWheelAngle_ ELKExit>"
  Bus Selector9/2 -> Bus Creator2/4  "<HWADATAClct_DriverBrakeHWAExit>"
  Bus Selector11/3 -> Bus Creator2/11  "<LDW_Con_SteerWheelAngle_ LDWExit>"
  Bus Selector11/13 -> Bus Creator2/21  "<ELK_Con_BrakePressure_ ELKExit>"
  Bus Selector8/1 -> Bus Creator2/1  "<ACCDataClct_ConNotStsf>"
  [ESS_DATA] -> Bus Selector15/1
  [EDR_ACCDataClct] -> Bus Selector8/1
  Bus Selector11/11 -> Bus Creator2/19  "<LKA_Con_OverRide_ LKAExit>"
  Bus Selector11/7 -> Bus Creator2/15  "<LKA_Con_BrakePressure_ LKAExit>"
  Bus Selector11/9 -> Bus Creator2/17  "<LKA_Con_DriverInput_ LKAExit>"
  [HWA_DATA] -> Bus Selector9/1
  Bus Selector15/2 -> Bus Creator2/31  "<ESSDataClct_DriverSteerESSExit>"
  Bus Selector9/1 -> Bus Creator2/3  "<HWADATAClct_OverrideHWAExit>"
  Bus Selector11/1 -> Bus Creator2/9  "<LDW_Con_AccPedalRate_LDWExit>"
  Bus Selector8/5 -> Bus Creator2/8  "<ACCDataClct_DriverSteerACCExit>"
  Bus Selector8/4 -> Bus Creator2/7  "<ACCDataClct_DriverBrakeACCExit>"
  Bus Selector11/15 -> Bus Creator2/23  "<ELK_Con_SteerWheelSpd_ ELKExit>"
  Bus Selector11/5 -> Bus Creator2/13  "<LDW_Con_SteerWheelSpd_ LDWExit>"
  Bus Selector11/2 -> Bus Creator2/10  "<LDW_Con_BrakePressure_ LDWExit>"
  Bus Selector15/1 -> Bus Creator2/30  "<ESSDataClct_OverrideESSExit>"
  Bus Selector11/16 -> Bus Creator2/24  "<LCK_Con_AccPedalRate_LCKExit>"
  Bus Selector8/3 -> Bus Creator2/6  "<ACCDataClct_OverrideACCExit>"
  Bus Selector11/20 -> Bus Creator2/28  "<LCK_Con_SteerWheelAngle_ LCKExit>"
  Bus Selector11/17 -> Bus Creator2/25  "<LCK_Con_BrakePress_ LCKExit>"
  Bus Selector11/18 -> Bus Creator2/26  "<LCK_Con_SteerAngleSpd_ LCKExit>"
  Bus Selector11/19 -> Bus Creator2/27  "<LCK_Con_OverRide_ LCKExit>"
  Bus Selector11/4 -> Bus Creator2/12  "<LDW_Con_DriverInput_ LDWExit>"
  Bus Selector11/21 -> Bus Creator2/29  "<LCK_Con_DriverInput_ LCKExit>"
  Bus Selector11/10 -> Bus Creator2/18  "<LKA_Con_SteerWheelSpd_ LKAExit>"
  [PilotSts] -> LSS/14(PilotSts)
  PLAN_NOH_SetSpdAdjVal/1 -> Cruise/17(PLAN_NOH_SetSpdAdjVal)
  PLAN_NOH_SetSpdAdjReq/1 -> Cruise/16(PLAN_NOH_SetSpdAdjReq)
  [VehConfig] -> ESS/7(VehConfig)
  [Diag] -> ESS/6(Dia)
  Cruise/5(HWA_TurnLightReq) -> [HWA_TurnLightReq]
  w4/1 -> TarDangerLevel/1  "TarDangerLevel"
  [HWA_TurnLightReq] -> HWA_TurnLightReq/1  "HWA_TurnLightReq"
  Signal Copy3/1 -> Bus Creator5/4  "RampDistance"
  Signal Copy2/1 -> Bus Creator5/3  "TunnelDistance"
  Signal Copy1/1 -> Bus Creator5/2  "FormOfWay"
  Signal Copy/1 -> Bus Creator5/1  "DrivingOnHighWay"
  Bus Selector14/4 -> Signal Copy3/1  "<f_start_distance>"
  Bus Selector14/3 -> Signal Copy2/1  "<f_tunnel_distance>"
  Bus Selector14/2 -> Signal Copy1/1  "<i_form_of_way>"
  Bus Selector14/1 -> Signal Copy/1  "<i_func_road_class>"
  EHRV2_ALL/1 -> Bus Selector14/1
  Bus Selector13/1 -> w118/1  "<HandsOffDetd>"
  [HODinfo] -> Bus Selector13/1
  EDR_HWAExit/1(HWA_DATA) -> [HWA_DATA]
  ESS/2(ESS_DATA) -> [ESS_DATA]
  [LSS_DATA] -> Bus Selector/1
  Cruise/3(EDR_ACCDataClct) -> [EDR_ACCDataClct]
  [IFC_Signal] -> Bus Selector7/1
  LSS/6(LSS_DATA) -> [LSS_DATA]
  [VSM_TSR_Init] -> TSR/6(VSM_TSR_Init)
  [AD_CAN] -> TSR/5(AD_CAN)
  [RF_input] -> TSR/4(RF_input)
  Unit Delay2/1 -> TSR/3(ISL_Actice)
  [Diag] -> TSR/2(Diag)
  [VehConfig] -> TSR/1(VehConfig)
  TSR/1(TSR_output) -> [TSR_output], Cruise/6(TSR_Info)
  [HWAStateInfo] -> Bus Selector6/1
  Compare To Constant6/1 -> w304/1
  Bus Selector19/14 -> Compare To Constant6/1  "<VSM_HWASts>"
  w35/1 -> HWASts/1  "HWASts"
  Bus Creator1/1 -> [EHR_Input]  "EHRV2_Input"
  Unit Delay4/1 -> HOD/3(LatStateInfo)
  Unit Delay3/1 -> HOD/2(HWAStateInfo)
  Unit Delay1/1 -> Cruise/1(LCKStateInfo)
  DriverSts/1 -> Switch6/1  "DriverSts"
  LSM_Cnt/1 -> Bus Creator/1  "LSM_Cnt"
  Bus Creator4/1 -> [Fusion_Line]
  Bus Creator/1 -> [Target_Line]
  Bus Creator5/1 -> Bus Creator1/1
  LSM_HWA/1 -> Bus Creator/3  "LSM_HWA"
  LSM_TJA_ICA/1 -> Bus Creator/2  "LSM_TJA_ICA"
  RFM_TSR/1 -> [RF_input]  "RFM_TSR"
  ESP_MasterCylBrkPressVld/1 -> Bus Creator3/31  "ESP_MasterCylBrkPressVld"
  CURRENT_GEAR/1 -> Bus Creator3/18  "CURRENT_GEAR"
  Ground5/1 -> Bus Creator3/9  "AccelPedalPosnVldty"
  EngState/1 -> Bus Creator3/11  "EngState"
  SHIFT_IN_PROGRESS/1 -> Bus Creator3/14  "SHIFT_IN_PROGRESS"
  EPS_LKATrqOvlDlvdSts/1 -> Bus Creator3/55  "EPS_LKATrqOvlDlvdSts"
  RLWheelSpd/1 -> Bus Creator3/47  "RLWheelSpd"
  PTCActv/1 -> Bus Creator3/34  "PTCActv"
  MSRActv/1 -> Bus Creator3/32  "MSRActv"
  BTCActv_RA/1 -> Bus Creator3/39  "BTCActv_RA"
  MSRActv_RA/1 -> Bus Creator3/37  "MSRActv_RA"
  ACAmbTemp/1 -> Bus Creator3/64  "ACAmbTemp"
  HazardLmpSwtSts/1 -> Bus Creator3/62  "HazardLmpSwtSts"
  DrvDoorSts/1 -> Bus Creator3/59  "DrvDoorSts"
  ESPFailSts/1 -> Bus Creator3/30  "ESPFailSts"
  PassengerDoorSts/1 -> Bus Creator3/60  "PassengerDoorSts"
  EPS_SteerMod/1 -> Bus Creator3/52  "EPS_SteerMod"
  HoodSts_F_Pbox/1 -> Bus Creator3/65  "HoodSts_F_Pbox"
  AccelPedalPosn/1 -> Bus Creator3/10  "AccelPedalPosn"
  RRWheelSpd/1 -> Bus Creator3/49  "RRWheelSpd"
  Bus Creator3/1 -> [AD_CAN]
  PTCActv_RA/1 -> Bus Creator3/38  "PTCActv_RA"
  EPS_LKATorqOvrlDlvd/1 -> Bus Creator3/53  "EPS_LKATorqOvrlDlvd"
  Switch5/1 -> Bus Creator3/27  "DrivingModDis"
  EPS_DrvInpTrqVal_HighReslolution/1 -> Bus Creator3/56  "EPS_DrvInpTrqVal_HighReslolution"
  ABSFailSts/1 -> Bus Creator3/40  "ABSFailSts"
  EngLimpHomeSts/1 -> Bus Creator3/12  "EngLimpHomeSts"
  TGS_LEVER/1 -> Bus Creator3/19  "TGS_LEVER"
  VehStandstill/1 -> Bus Creator3/22  "VehStandstill"
  HDCCtrl/1 -> Bus Creator3/23  "HDCCtrl"
  VehSpd/1 -> Bus Creator3/42  "VehSpd"
  TargetGearValid/1 -> Bus Creator3/15  "TargetGearValid"
  SysPowerMod/1 -> Bus Creator3/57  "SysPowerMod"
  RFM_LINE_R1/1 -> Bus Creator4/2  "RFM_LINE_R1"
  ESP_MasterCylBrkPress/1 -> Bus Creator3/36  "ESP_MasterCylBrkPress"
  WiprReq/1 -> Bus Creator3/58  "WiprReq"
  EPBSts/1 -> Bus Creator3/44  "EPBSts"
  TARGET_GEAR/1 -> Bus Creator3/16  "TARGET_GEAR"
  CDDAvailable/1 -> Bus Creator3/25  "CDDAvailable"
  ECMRespACC/1 -> Bus Creator3/7  "ECMRespACC"
  VDCActv/1 -> Bus Creator3/33  "VDCActv"
  NoBrkForce/1 -> Bus Creator3/21  "NoBrkForce"
  EPB_SwtPosn/1 -> Bus Creator3/45  "EPB_SwtPosn"
  WindshldWiprActvSts/1 -> Bus Creator3/61  "WindshldWiprActvSts"
  "KL30BRelaySts "/1 -> Bus Creator3/63  "KL30BRelaySts"
  EngSpd/1 -> Bus Creator3/2  "EngSpd"
  ESPBrkLmpCtrl/1 -> Bus Creator3/29  "ESPBrkLmpCtrl"
  Switch/1 -> Bus Creator3/1  "BrkPedalSts"
  ESPFuncOffSts/1 -> Bus Creator3/28  "ESPFuncOffSts"
  Switch1/1 -> Bus Creator3/4  "AccPedalOverride"
  AVHSts/1 -> Bus Creator3/26  "AVHSts"
  EPS_TrqSnsrSts/1 -> Bus Creator3/51  "EPS_TrqSnsrSts"
  CAL_VSM_CONFIG/1 -> [VehConfig]  "CAL_VSM_CONFIG"
  ShiftInPrgValid/1 -> Bus Creator3/17  "ShiftInPrgValid"
  Switch3/1 -> Bus Creator3/8  "ECMACCInterface"
  Start_StopSts/1 -> Bus Creator3/3  "Start_StopSts"
  CDDActv/1 -> Bus Creator3/24  "CDDActv"
  EBDFailSts/1 -> Bus Creator3/41  "EBDFailSts"
  RFM_LINE_L1/1 -> Bus Creator4/1  "RFM_LINE_L1"
  EPS_FailSts/1 -> Bus Creator3/50  "EPS_FailSts"
  RRWheelDriveDirection/1 -> Bus Creator3/48  "RRWheelDriveDirection"
  BrkDskOvrheatd/1 -> Bus Creator3/20  "BrkDskOvrheatd"
  BTCActv/1 -> Bus Creator3/35  "BTCActv"
  EPS_LKATorqOvrlDlvdVld/1 -> Bus Creator3/54  "EPS_LKATorqOvrlDlvdVld"
  RLWheelDriveDirection/1 -> Bus Creator3/46  "RLWheelDriveDirection"
  CurrentGearValid/1 -> Bus Creator3/13  "CurrentGearValid"
  Switch2/1 -> Bus Creator3/6  "AccelPedlPosnDiagc"
  ABSActv/1 -> Bus Creator3/43  "ABSActv"
  epsTrqReqValue/1 -> Bus Creator12/1  "epsTrqReqValue"
  epsTrqReqFlag/1 -> Bus Creator12/2  "epsTrqReqFlag"
  Bus Creator12/1 -> [BusLatCtrlInfo]
  kapTraj/1 -> Bus Creator19/6  "kapTraj"
  ayvRefMs2/1 -> Bus Creator19/5  "ayvRefMs2"
  AEB_VehResp/1 -> Bus Creator19/7  "AEB_VehResp"
  psiDtOpt/1 -> Bus Creator19/4  "psiDtOpt"
  AEB_PedResp/1 -> Bus Creator19/8  "AEB_PedResp"
  axvRoadSlopeMs2/1 -> Bus Creator19/3  "axvRoadSlopeMs2"
  vxvRefMs/1 -> Bus Creator19/2  "vxvRefMs"
  axvRefMs2/1 -> Bus Creator19/1  "axvRefMs2"
  Bus Creator19/1 -> [VehicleSts]
  DFIM_VSM_STS/1 -> [Diag]  "DFIM_VSM_STS"
  VSM_TSR_INIT/1 -> [VSM_TSR_Init]  "SPL_noSupp_Dist_Init"
  RFM_LINEF_LB/1 -> Bus Creator4/3  "RFM_LINEF_LB"
  RFM_LINEF_RB/1 -> Bus Creator4/4  "RFM_LINEF_RB"
  LSM_ESS/1 -> Bus Creator/5  "LSM_ESS"
  LSM_LCK/1 -> Bus Creator/4  "LSM_LCK"
  DriveOffConditionFulfilled/1 -> Bus Creator19/13  "DriveOffConditionFulfilled"
  TOS_ACCP0/1 -> [ACC_P0]  "TOS_ACCP0"
  FFogLmpSts_F_Pbox/1 -> Bus Creator3/66  "FFogLmpSts_F_Pbox"
  RFogLmpSts_R_Pbox/1 -> Bus Creator3/67  "RFogLmpSts_R_Pbox"
  LowBeamSts/1 -> Bus Creator3/68  "LowBeamSts"
  SteerWheelAngSign/1 -> Bus Creator3/74  "SteerWheelAngSign"
  SteerWheelSpd/1 -> Bus Creator3/75  "SteerWheelSpd"
  FrntWiprSwtSts/1 -> Bus Creator3/70  "FrntWiprSwtSts"
  RTurnLmpSwtSts/1 -> Bus Creator3/72  "RTurnLmpSwtSts"
  LTurnLmpSwtSts/1 -> Bus Creator3/71  "LTurnLmpSwtSts"
  FrntWshrSwtSts/1 -> Bus Creator3/69  "FrntWshrSwtSts"
  SteerWheelAng/1 -> Bus Creator3/73  "SteerWheelAng"
  IP_VehSpdUnit/1 -> Bus Creator3/91  "IP_VehSpdUnit"
  OR1/1 -> Bus Creator3/94  "LCKSwtReq"
  VehLatAccel/1 -> Bus Creator3/89  "VehLatAccel"
  CC_ACC_CANCEL_OFFSwt/1 -> Bus Creator3/81  "CC_ACC_CANCEL_OFFSwt"
  CC_ACC_DecSetSpd_SetSwt/1 -> Bus Creator3/83  "CC_ACC_DecSetSpd_SetSwt"
  DrvSBR/1 -> Bus Creator3/86  "DrvSBR"
  ACC_TimeGap_DecSetSwt/1 -> Bus Creator3/79  "ACC_TimeGap_DecSetSwt"
  PassSBR/1 -> Bus Creator3/87  "PassSBR"
  CC_ACC_IncSetSpd_ResuSwt/1 -> Bus Creator3/82  "CC_ACC_IncSetSpd_ResuSwt"
  VehLgtAccel/1 -> Bus Creator3/88  "VehLgtAccel"
  VehYawRate/1 -> Bus Creator3/90  "VehYawRate"
  IFC_SnvtySet/1 -> Bus Creator3/92  "IFC_SnvtySet"
  HWA_OK_OFFSwt/1 -> Bus Creator3/85  "HWA_OK_OFFSwt"
  CC_ACCSwtErr/1 -> Bus Creator3/84  "CC_ACCSwtErr"
  SAS_Sts/1 -> Bus Creator3/77  "SAS_Sts"
  OR/1 -> Bus Creator3/93  "LKASwtReq"
  ACC_TimeGap_IncSetSwt/1 -> Bus Creator3/78  "ACC_TimeGap_IncSetSwt"
  SteerWheelSpdSign/1 -> Bus Creator3/76  "SteerWheelSpdSign"
  CC_ACC_CRUISE_OFFSwt/1 -> Bus Creator3/80  "CC_ACC_CRUISE_OFFSwt"
  OR5/1 -> Bus Creator3/98  "LDWSwtReq"
  OR2/1 -> Bus Creator3/95  "ELKSwtReq"
  ALC_SwtReq/1 -> Bus Creator3/110  "ALC_SwtReq"
  OR9/1 -> Bus Creator3/102  "ISLSwtReq"
  OR14/1 -> Bus Creator3/105  "LSSSwtReq"
  OR8/1 -> Bus Creator3/101  "ICA_HandsOffSwtReq"
  OR7/1 -> Bus Creator3/100  "TSRWarnSwtReq"
  OR6/1 -> Bus Creator3/99  "TSRSwtReq"
  OR4/1 -> Bus Creator3/97  "ESS_VehSwtReq"
  HWA_SwtReq/1 -> Bus Creator3/108  "HWA_SwtReq"
  OR12/1 -> Bus Creator3/107  "AESSwtReq"
  OR15/1 -> Bus Creator3/106  "IntelligentEvaSwtReq"
  DVRWorkSts/1 -> Bus Creator3/130  "DVRWorkSts"
  APS_WorkSts/1 -> Bus Creator3/129  "APS_WorkSts"
  CR_BrkgReq/1 -> Bus Creator3/114  "CR_BrkgReq"
  HighBeamSts/1 -> Bus Creator3/115  "HighBeamSts"
  USS_FrontSys_Status/1 -> Bus Creator3/116  "USS_FrontSys_Status"
  USS_FLCNear_Obj_Pos_X/1 -> Bus Creator3/118  "USS_FLCNear_Obj_Pos_X"
  USS_FLCNear_Obj_Pos_Y/1 -> Bus Creator3/119  "USS_FLCNear_Obj_Pos_Y"
  USS_FLCNear_Obj_Confidence/1 -> Bus Creator3/117  "USS_FLCNear_Obj_Confidence"
  USS_FLMNear_Obj_Pos_Y/1 -> Bus Creator3/122  "USS_FLMNear_Obj_Pos_Y"
  USS_FLMNear_Obj_Confidence/1 -> Bus Creator3/120  "USS_FLMNear_Obj_Confidence"
  USS_FRCNear_Obj_Pos_X/1 -> Bus Creator3/127  "USS_FRCNear_Obj_Pos_X"
  USS_FRCNear_Obj_Pos_Y/1 -> Bus Creator3/128  "USS_FRCNear_Obj_Pos_Y"
  USS_FRMNear_Obj_Pos_X/1 -> Bus Creator3/124  "USS_FRMNear_Obj_Pos_X"
  USS_FRMNear_Obj_Pos_Y/1 -> Bus Creator3/125  "USS_FRMNear_Obj_Pos_Y"
  USS_FRMNear_Obj_Confidence/1 -> Bus Creator3/123  "USS_FRMNear_Obj_Confidence"
  USS_FLMNear_Obj_Pos_X/1 -> Bus Creator3/121  "USS_FLMNear_Obj_Pos_X"
  USS_FRCNear_Obj_Confidence/1 -> Bus Creator3/126  "USS_FRCNear_Obj_Confidence"
  IFCHUTInterface/1 -> Bus Creator1/2  "IFCHUTInterface"
  MapDataValid/1 -> Bus Creator1/3  "MapDataValid"
  " "/1 -> Bus Creator19/12  "AEB_TgtDecel_Req"
  Inter_FCW_Warn/1 -> Bus Creator19/9  "Inter_FCW_Warn"
  TOS_ELK/1 -> [ELK_Obj]  "ELK_Object_Fus_Type"
  TOS_LCKIE/1 -> [LCKIE_Obj]  "TOS_LCKIE"
  TOS_AEB_LONOBJ_BUS/1 -> [AEB_OBJ]
  AEB_VehTrig/1 -> Bus Creator19/10  "AEB_VehTrig"
  AEB_PedTrig/1 -> Bus Creator19/11  "AEB_PedTrig"
  HCU_GearSts/1 -> Bus Creator3/131
  HCU_PTDrvMod/1 -> Terminator9/1
  ACU_ShiftInProgress/1 -> Terminator8/1
  [LatStateInfo] -> LSMC_Debug/1
  [LCKStateInfo] -> LCK_Debugold/1
  w431/1 -> TarLineC3/1  "TarLineC3"
  Bus Selector19/7 -> w35/1  "<VSM_HWASts>"
  Bus Selector20/2 -> w372/1  "<ISL_InterSysInfoDisp>"
  tt9/1 -> AESSts/1  "AESSts"
  Bus Selector76/21 -> Bus Creator8/21  "<VSM_HWAFastExitCons_ACCNotActive>"
  [HWAStateInfo] -> Bus Selector63/1
  w447/1 -> ELKLineRange/1  "ELKLineRange"
  Bus Selector10/2 -> TSRResp/1  "<TSRResp>"
  Bus Selector75/11 -> Bus Creator7/11  "<VSM_ACCFastExitCons_DriverDoorOpen>"
  Bus Selector10/12 -> TSRTrfcSignVal/1  "<TSRTrfcSignVal>"
  MATLAB Function2/1(DriverInloop_Monitor) -> w463/1  "DriverInloop_Monitor"
  Bus Selector23/1 -> w117/1  "<VSM_HWAWarningLevel>"
  Bus Selector57/1 -> w460/1  "<ALC_SwtReq>"
  Bus Selector76/11 -> Bus Creator8/11  "<VSM_ACCSlowExitCons_HDCactive40ms>"
  Bus Selector76/41 -> Bus Creator8/41  "<VSM_HWAActivationCons_NoHWANoError>"
  Bus Selector24/1 -> w119/1  "<TJA_ACC_SelSts>"
  From16/1 -> Bus Selector76/1, Bus Selector75/1
  [HWAStateInfo] -> Bus Selector20/1
  w33/1 -> ACC_ParkShiftReq/1  "ACC_ParkShiftReq"
  [DriverSts] -> MATLAB Function2/1(DriverSts)
  Bus Selector19/1 -> w449/1  "<Signal_ACC_ModeSts>"
  Bus Selector75/3 -> Bus Creator7/3  "<VSM_ACCFastExitCons_RollingBack>"
  Bus Selector10/11 -> TSRConSpdLimWarn/1  "<TSRConSpdLimWarn>"
  Bus Selector76/52 -> Bus Creator8/52  "<DriverStsGood>"
  w435/1 -> TarLineRange/1  "TarLineRange"
  w445/1 -> ELKLineC1/1  "ELKLineC1"
  w106/1 -> CruiseChauffeur_ModeDisp/1  "CruiseChauffeur_ModeDisp"
  Bus Selector19/2 -> w37/1  "<Signal_ACC_SpdSetValue>"
  w430/1 -> TarLineValid/1  "TarLineValid"
  Bus Selector75/5 -> Bus Creator7/5  "<VSM_ACCFastExitCons_BrakeDiskOverHeat>"
  Bus Selector19/16 -> w107/1  "<Signal_ACCTextDisp>"
  Bus Selector22/2 -> w431/1  "<VSM_TarLineC3>"
  w449/1 -> ACCSts/1  "ACCSts"
  w439/1 -> LKALineC1/1  "LKALineC1"
  Bus Selector10/8 -> TSRSpdLimCfdc/1  "<TSRSpdLimCfdc>"
  Bus Selector22/1 -> w430/1  "<VSM_TarLineValid>"
  Bus Selector19/13 -> w289/1  "<Signal_HWAModeDisp>"
  [Control_Lane] -> Bus Selector22/1
  Bus Selector76/2 -> Bus Creator8/2  "<VSM_HWASlowExitCons_AEBOff>"
  w442/1 -> ELKLineValid/1  "ELKLineValid"
  Bus Selector47/3 -> w453/1  "<LKAWarning>"
  w39/1 -> ACC_TimeGapSet/1  "ACC_TimeGapSet"
  Bus Selector76/51 -> Bus Creator8/51  "<HazardLmpSwtStsOff>"
  Bus Selector20/1 -> w371/1  "<ISL_Resp>"
  Bus Selector76/48 -> Bus Creator8/48  "<HWANoError>"
  Bus Selector10/20 -> SPL_SuppName_Value_Remain/1  "<SPL_SuppName_Value_Remain>"
  Bus Selector76/7 -> Bus Creator8/7  "<VSM_HWASlowExitCons_DVRError>"
  Bus Selector76/27 -> Bus Creator8/27  "<VSM_HWAActivationCons_VehicleSpdNormal3s>"
  w41/1 -> ACC_ModeDisp/1  "ACC_ModeDisp"
  w453/1 -> LKAWarning/1  "LKAWarning"
  Bus Selector76/9 -> Bus Creator8/9  "<VSM_ACCSlowExitCons_EspActive400ms>"
  Bus Selector22/4 -> w433/1  "<VSM_TarLineC1>"
  [ELK_Lane] -> Bus Selector46/1
  Bus Selector76/35 -> Bus Creator8/35  "<VSM_HWAActivationCons_NoDoubleLineLost>"
  [LatStateInfo] -> Bus Selector2/1
  Bus Selector76/47 -> Bus Creator8/47  "<MapDataValid>"
  Bus Selector10/10 -> TSRConSpdLim/1  "<TSRConSpdLim>"
  Bus Selector76/39 -> Bus Creator8/39  "<VSM_HWAActivationCons_MapDataValid>"
  Bus Creator8/1 -> HWAExitConds/1  "HWAExitConds"
  w461/1 -> HWA_LaneChangeReq/1  "HWA_LaneChangeReq"
  w441/1 -> LKALineRange/1  "LKALineRange"
  Bus Selector10/14 -> SPL_noSupp_Dist_Remain/1  "<SPL_noSupp_Dist_Remain>"
  Bus Selector76/24 -> Bus Creator8/24  "<VSM_HWAFastExitCons_StandstillTimeout>"
  Bus Selector75/9 -> Bus Creator7/9  "<VSM_ACCFastExitCons_DriveBrakeExit>"
  [IFC_Signal] -> Bus Selector1/1
  Bus Selector76/49 -> Bus Creator8/49  "<LTurnLightSwOff>"
  w436/1 -> LKALineValid/1  "LKALineValid"
  Bus Selector76/28 -> Bus Creator8/28  "<VSM_HWAActivationCons_TJAActive>"
  Bus Selector10/7 -> TSRSpdLim/1  "<TSRSpdLim>"
  Bus Selector46/1 -> w442/1  "<VSM_ELKLaneValid>"
  w315/1 -> TJATextDisp/1  "TJATextDisp"
  w448/1 -> ISLActive/1  "ISLActive"
  Bus Selector76/37 -> Bus Creator8/37  "<VSM_HWAActivationCons_NoTunnel300m>"
  Bus Selector19/17 -> w315/1  "<Signal_TJATextDisp>"
  w3/1 -> HWATextDisp/1  "HWATextDisp"
  w444/1 -> ELKLineC2/1  "ELKLineC2"
  Bus Selector20/3 -> w448/1  "<ISL_Active>"
  Bus Creator7/1 -> ACCExitConds/1  "ACCExitConds"
  Bus Selector75/7 -> Bus Creator7/7  "<VSM_ACCFastExitCons_EspOff>"
  Bus Selector43/2 -> w437/1  "<VSM_LKALaneA3>"
  Bus Selector76/10 -> Bus Creator8/10  "<VSM_ACCSlowExitCons_MSRactive800ms>"
  w443/1 -> ELKLineC3/1  "ELKLineC3"
  Bus Selector10/5 -> TSRSpdLimUnit/1  "<TSRSpdLimUnit>"
  Bus Selector76/33 -> Bus Creator8/33  "<VSM_HWAActivationCons_HWALineValid>"
  Bus Selector19/10 -> w41/1  "<Signal_ACC_ModDisp>"
  w460/1 -> ALC_Resp/1  "ALC_Resp"
  Bus Selector19/9 -> w38/1  "<Signal_ACC_HazActv>"
  Bus Selector76/44 -> Bus Creator8/44  "<DoubleLineNotLostOrP0TargetExist>"
  Bus Selector76/6 -> Bus Creator8/6  "<VSM_HWASlowExitCons_MapDataInvalid>"
  Bus Selector46/3 -> w444/1  "<VSM_ELKLaneA2>"
  Bus Selector10/1 -> TSRSts/1  "<TSRSts>"
  Bus Selector22/3 -> w432/1  "<VSM_TarLineC2>"
  Bus Selector76/3 -> Bus Creator8/3  "<VSM_HWASlowExitCons_HandsoffOverride>"
  Bus Selector75/10 -> Bus Creator7/10  "<VSM_ACCFastExitCons_EPBClosed>"
  w463/1 -> DriverInloop_Monitor/1  "DriverInloop_Monitor"
  Bus Selector76/53 -> Bus Creator8/53  "<AEBSwitchOn>"
  w372/1 -> ISL_InterSysInfoDisp/1  "ISL_InterSysInfoDisp"
  Bus Selector76/42 -> Bus Creator8/42  "<VSM_HWAActivationCons_NoHWASafeStopHappened_b>"
  Bus Selector75/8 -> Bus Creator7/8  "<VSM_ACCFastExitCons_NoForwardGear>"
  Bus Selector75/13 -> Bus Creator7/13  "<VSM_ACCSlowExitCons_MSRactive800ms>"
  w34/1 -> TJASts/1  "TJASts"
  Bus Selector76/23 -> Bus Creator8/23  "<VSM_HWAFastExitCons_ParkGearOrEPBActive>"
  w40/1 -> ACC_DrvOffReq/1  "ACC_DrvOffReq"
  Bus Selector76/40 -> Bus Creator8/40  "<VSM_HWAActivationCons_DVRNoError>"
  Bus Selector76/18 -> Bus Creator8/18  "<VSM_HWASlowExitCons_HWAError_Inhibit>"
  Bus Selector76/31 -> Bus Creator8/31  "<VSM_HWAActivationCons_DriverStsGood10s>"
  Bus Selector76/15 -> Bus Creator8/15  "<VSM_ACCFastExitCons_DriverSBR>"
  Bus Selector75/4 -> Bus Creator7/4  "<VSM_ACCFastExitCons_EngineOff>"
  Bus Selector22/5 -> w434/1  "<VSM_TarLineC0>"
  w42/1 -> TJA_ModeDisp/1  "TJA_ModeDisp"
  Bus Selector75/1 -> Bus Creator7/1  "<VSM_ACCFastExitCons_Standstill3min>"
  Bus Selector76/13 -> Bus Creator8/13  "<VSM_ACCSlowExitCons_TCS1active3000ms>"
  Bus Selector76/25 -> Bus Creator8/25  "<VSM_HWAFastExitCons_OverrideTimeout>"
  Bus Selector76/45 -> Bus Creator8/45  "<DrivingOnHighWay>"
  [TSR_output] -> Bus Selector10/1
  w157/1 -> ICA_HandsOffSwtResp/1  "ICA_HandsOffSwtResp"
  Bus Selector76/32 -> Bus Creator8/32  "<VSM_HWAActivationCons_AEBSwitchOn>"
  w119/1 -> TJA_ACC_SelSts/1  "TJA_ACC_SelSts"
  Bus Selector76/29 -> Bus Creator8/29  "<VSM_HWAActivationCons_LCKActive>"
  w446/1 -> ELKLineC0/1  "ELKLineC0"
  w464/1 -> LaneAvailability/1  "LaneAvailability"
  Bus Selector76/26 -> Bus Creator8/26  "<VSM_HWAFastExitCons_SpeedTooHighWithOverride>"
  Bus Selector19/3 -> w39/1  "<Signal_ACC_TimeGapSet>"
  w371/1 -> ACC_ISLResp/1  "ACC_ISLResp"
  Bus Selector75/14 -> Bus Creator7/14  "<VSM_ACCSlowExitCons_HDCactive40ms>"
  Bus Selector76/16 -> Bus Creator8/16  "<VSM_HWASlowExitCons_NotHighWayArterialRoad5s>"
  Bus Selector1/1 -> w110/1  "<Signal_HandsOffWarn>"
  Bus Selector57/4 -> w157/1  "<ICA_HandsOffSwtReq>"
  MATLAB Function4/1(HWAAccControlSts) -> w466/1  "HWAAccControlSts"
  w452/1 -> ELKSts/1  "ELKSts"
  Bus Selector43/3 -> w438/1  "<VSM_LKALaneA2>"
  [DriverSts] -> MATLAB Function4/3(DriverSts)
  w459/1 -> HWA_SnvtySet_Resp/1  "HWA_SnvtySet_Resp"
  [ESSState] -> w32/1  "ESSSts"
  w465/1 -> TJA_FollowSts/1  "TJA_FollowSts"
  Bus Selector76/50 -> Bus Creator8/50  "<RTurnLightSwOff>"
  w115/1 -> LCKSts/1  "LCKSts"
  Bus Selector46/6 -> w447/1  "<VSM_ELKLaneRange>"
  Bus Selector46/2 -> w443/1  "<VSM_ELKLaneA3>"
  Bus Selector76/34 -> Bus Creator8/34  "<VSM_HWAActivationCons_NoSingleLineLost>"
  Bus Selector76/8 -> Bus Creator8/8  "<VSM_HWASlowExitCons_SingleLineLost>"
  Bus Selector46/5 -> w446/1  "<VSM_ELKLaneA0>"
  w32/1 -> ESSSts/1  "ESSSts"
  Bus Selector63/2 -> MATLAB Function4/2(TJASts)  "<TJASts>"
  Bus Selector19/6 -> w34/1  "<TJASts>"
  Bus Selector10/3 -> TSRWarnResp/1  "<TSRWarnResp>"
  Bus Selector46/4 -> w445/1  "<VSM_ELKLaneA1>"
  Bus Selector76/30 -> Bus Creator8/30  "<VSM_HWAActivationCons_HandsOn5s>"
  w466/1 -> HWAAccControlSts/1  "HWAAccControlSts"
  Bus Selector76/46 -> Bus Creator8/46  "<FormOfWay>"
  Bus Selector76/38 -> Bus Creator8/38  "<VSM_HWAActivationCons_NoForkRoad300m>"
  Bus Selector76/1 -> Bus Creator8/1  "<VSM_HWASlowExitCons_AEBTrigger>"
  Bus Selector75/16 -> Bus Creator7/16  "<VSM_ACCSlowExitCons_TCS1active3000ms>"
  w36/1 -> HWAActive/1  "HWAActive"
  Bus Selector10/17 -> SPL_noSupp_Value_Remain/1  "<SPL_noSupp_Value_Remain>"
  Bus Selector10/15 -> SPL_whSupp_Dist_Remain/1  "<SPL_whSupp_Dist_Remain>"
  w450/1 -> LKASts/1  "LKASts"
  w437/1 -> LKALineC3/1  "LKALineC3"
  Bus Selector19/11 -> w33/1  "<Signal_ACC_ParkShiftReq>"
  w451/1 -> LDWSts/1  "LDWSts"
  [LKA_Lane] -> Bus Selector43/1
  [HWAStateInfo] -> Bus Selector24/1
  w438/1 -> LKALineC2/1  "LKALineC2"
  [AD_CAN] -> Bus Selector57/1
  Bus Selector76/36 -> Bus Creator8/36  "<VSM_HWAActivationCons_HighWayArterialRoad>"
  w107/1 -> ACCTextDisp/1  "ACCTextDisp"
  Bus Selector10/19 -> TS_SignName_Value_Remain/1  "<TS_SignName_Value_Remain>"
  Bus Selector76/17 -> Bus Creator8/17  "<VSM_HWASlowExitCons_LCKIdleWithoutTurnLight>"
  Bus Selector2/1 -> w115/1  "<LCK_State>"
  Bus Selector19/8 -> w36/1  "<VSM_HWAActive>"
  w434/1 -> TarLineC0/1  "TarLineC0"
  Bus Selector43/5 -> w440/1  "<VSM_LKALaneA0>"
  w462/1 -> LSS_WarnFormSwtResp/1  "LSS_WarnFormSwtResp"
  Bus Selector75/17 -> Bus Creator7/17  "<VSM_ACCSlowExitCons_TCS2active3000ms>"
  Bus Selector10/6 -> TSRSpdLimSts/1  "<TSRSpdLimSts>"
  Bus Selector76/22 -> Bus Creator8/22  "<VSM_HWAFastExitCons_HWAErrorFastExit>"
  Bus Selector10/13 -> TSRTrfcSignValCfdc/1  "<TSRTrfcSignValCfdc>"
  w12/1 -> AND/1  "ACC_SOS_Req"
  [AD_CAN] -> Bus Selector60/1
  w37/1 -> ACC_SpdSetValue/1  "ACC_SpdSetValue"
  Bus Selector75/2 -> Bus Creator7/2  "<VSM_ACCFastExitCons_StandstillNoBrakeForce>"
  Bus Selector76/19 -> Bus Creator8/19  "<VSM_HWASlowExitCons_HWAError_Error>"
  Bus Selector63/1 -> MATLAB Function4/1(HWASts)  "<VSM_HWASts>"
  Bus Selector22/6 -> w435/1  "<VSM_TarLineRange>"
  Bus Selector75/6 -> Bus Creator7/6  "<VSM_ACCFastExitCons_Cancel>"
  Bus Selector43/6 -> w441/1  "<VSM_LKALaneRange>"
  Bus Selector10/18 -> SPL_whSupp_Value_Remain/1  "<SPL_whSupp_Value_Remain>"
  w117/1 -> HWA_Warning/1  "HWA_Warning"
  Bus Selector19/12 -> w42/1  "<Signal_TJA_ModeSts>"
  Bus Selector76/4 -> Bus Creator8/4  "<VSM_HWASlowExitCons_HighSpdIn3s>"
  Bus Selector60/1 -> w462/1  "<LSSWarnFormSwtReq>"
  Bus Selector47/4 -> w452/1  "<ELK_State>"
  w289/1 -> HWA_ModeDisp/1  "HWA_ModeDisp"
  Bus Selector19/15 -> w106/1  "<Signal_CruiseChauffer_Sts>"
  w108/1 -> CCTextDisp/1  "CCTextDisp"
  tt8/1 -> EPBTakeOver_Req/1  "EPBTakeOver_Req"
  w432/1 -> TarLineC2/1  "TarLineC2"
  w304/1 -> HWASlowRetreat_b/1  "HWASlowRetreat_b"
  w116/1 -> vSetBelowMin/1  "vSetBelowMin"
  Bus Selector43/1 -> w436/1  "<VSM_LKALaneValid>"
  Bus Selector57/3 -> w13/1  "<HWA_SwtReq>"
  Bus Selector76/20 -> Bus Creator8/20  "<VSM_HWASlowExitCons_HWAError_ErrorBlindness>"
  Bus Selector10/9 -> TSRSpdLimWarn/1  "<TSRSpdLimWarn>"
  Bus Selector7/1 -> w464/1  "<LaneAvaliability>"
  [HWAStateInfo] -> Bus Selector23/1
  Bus Selector19/5 -> w40/1  "<Signal_ACC_DrvOFF_Req>"
  Bus Selector57/2 -> w459/1  "<HWA_SnvtySet>"
  [HWAStateInfo] -> Bus Selector19/1
  Bus Selector10/4 -> TSR_Snvty/1  "<TSR_Snvty>"
  Bus Selector47/1 -> w451/1  "<LDW_State>"
  [DangerPlausMatrix] -> DangerPlausMatrix/1
  Bus Selector75/15 -> Bus Creator7/15  "<VSM_ACCSlowExitCons_ABSactive400ms>"
  Bus Selector76/5 -> Bus Creator8/5  "<VSM_HWASlowExitCons_DMSInvalid>"
  w38/1 -> ACC_HazActv/1  "ACC_HazActv"
  Bus Selector22/7 -> w4/1  "<VSM_TarDangerLevel>"
  Bus Selector76/43 -> Bus Creator8/43  "<VSM_HWAActivationCons_NoHWAFastExitConditions_b>"
  w110/1 -> HandsOffWarningLevel/1  "HandsOffWarningLevel"
  Bus Selector76/12 -> Bus Creator8/12  "<VSM_ACCSlowExitCons_ABSactive400ms>"
  w118/1 -> HandsOffDetd/1  "HandsOffDetd"
  Bus Selector75/12 -> Bus Creator7/12  "<VSM_ACCSlowExitCons_EspActive400ms>"
  Bus Selector10/16 -> TS_SignName_Dist_Remain/1  "<TS_SignName_Dist_Remain>"
  w13/1 -> HWA_Resp/1
  Bus Selector19/4 -> w116/1  "<vSetBelowMin>"
  Bus Selector47/2 -> w450/1  "<LKA_State>"
  Bus Selector75/18 -> Bus Creator7/18  "<VSM_ACCFastExitCons_DriverSBR>"
  Bus Selector47/5 -> w454/1  "<LCKIE_Laneoffset>"
  w433/1 -> TarLineC1/1  "TarLineC1"
  [LatStateInfo] -> Bus Selector47/1
  w454/1 -> LCKIEDist/1  "LCKIEDist"
  Bus Selector76/14 -> Bus Creator8/14  "<VSM_ACCSlowExitCons_TCS2active3000ms>"
  w440/1 -> LKALineC0/1  "LKALineC0"
  Bus Selector43/4 -> w439/1  "<VSM_LKALaneA1>"
  Longctrl_Decel_ReqValue/1 -> Bus Creator19/14  "Longctrl_Decel_ReqValue"
  Bus Selector4/1 -> w1/1  "<LCKIE_State>"
  [LatStateInfo] -> Bus Selector4/1
  w1/1 -> LCKIESts/1  "LCKIESts"
  Constant4/1 -> Compare To Constant/1
  Compare To Constant/1 -> [Config_ICE_PHEV]
  [Config_ICE_PHEV] -> Switch/2
  BrkPedalSts/1 -> Switch/1
  HCU_BrkPedalSts/1 -> Switch/3
  [Config_ICE_PHEV] -> Switch1/2
  DrvTrqReqOvld/1 -> Switch1/3
  AccPedalOverride/1 -> Switch1/1
  HCU_PowertrainSts/1 -> Bus Creator3/5
  [Config_ICE_PHEV] -> Switch2/2
  HCU_AccelPedalPosn_Diag/1 -> Switch2/3
  AccelPedlPosnDiagc/1 -> Switch2/1
  [Config_ICE_PHEV] -> Switch3/2
  HCU_ACCInterface/1 -> Switch3/3
  ECMACCInterface/1 -> Switch3/1
  EngState_PHEV/1 -> Terminator/1  "EngState"
  [Config_ICE_PHEV] -> Switch5/2
  HCU_DrvMod/1 -> Direct Lookup Table (n-D)/1
  DrivingModDis/1 -> Switch5/1
  Bus Selector19/19 -> w2/1  "<SetSpeedKmH>"
  Bus Selector/1 -> EDR_HWAExit/4(<VSM_LCK_Con_SteerAngleSpd_Active2Ready>)  "<LCK_Con_SteerAngleSpd_ LCKExit>"
  Bus Selector3/1 -> EDR_HWAExit/2(<EDR_DriverBrakeHWAExit>)  "<EDR_DriverBrakeHWAExit>"
  HOD/1(HODinfo) -> Cruise/15(HODinfo), LSS/4(HODinfo), [HODinfo]
  LSS/1(LatStateInfo) -> [LatStateInfo], Unit Delay1/1  "LCKStateInfo"
  [EHR_Input] -> Cruise/8(EHR_Input)
  ESS/1(VSM_ESSState) -> [ESSState], LSS/5(ESSSts)
  Bus Selector/2 -> EDR_HWAExit/5(<VSM_LCK_Con_OverRide_Active2Ready>), OR10/1  "<LCK_Con_OverRide_ LCKExit>"
  Bus Selector/4 -> EDR_HWAExit/7(<VSM_LCK_Con_DriverInput_Active2Ready>), OR10/2  "<LCK_Con_DriverInput_ LCKExit>"
  [VehicleSts] -> Cruise/10(VehicleSts)
  [AD_CAN] -> LSS/13(AD_CAN)
  Bus Selector21/1 -> EDR_HWAExit/3(<EDR_OverrideHWAExit>)  "<ACCDataClct_OverrideACCExit>"
  [Target_Line] -> LSS/6(Target_Line)
  LSS/3(Control_Lane) -> [Control_Lane]
  [ACC_P0] -> LSS/12(ACC_P0)
  [LCKIE_Obj] -> LSS/9(LCKIE_Obj)
  Bus Selector6/1 -> EDR_HWAExit/1(HWAActive_b)  "<VSM_HWAActive>"
  [EDR_Longitude_HWAExit] -> Bus Selector3/1
  LSS/2(IFC_Signal) -> [IFC_Signal]
  [VehicleSts] -> LSS/8(VehicleSts)
  [Target_Line] -> ESS/4(Target_Line)
  LSS/5(LKA_Lane) -> [LKA_Lane]
  [VehConfig] -> LSS/2(VehConfig)
  [Diag] -> Cruise/5(Diag)
  ALC/1 -> Cruise/2(ALC), [ALC]
  LSS/4(ELK_Lane) -> [ELK_Lane]
  [Diag] -> LSS/3(Diag)
  Bus Selector/3 -> EDR_HWAExit/6(<VSM_LCK_Con_SteerWheelAngle_Active2Ready>)  "<LCK_Con_SteerWheelAngle_ LCKExit>"
  [AD_CAN] -> Cruise/11(AD_CAN)
  Cruise/4(HWAStateInfo) -> [HWAStateInfo], LSS/1(HWAStateInfo)
  [ACC_P0] -> Cruise/9(ACC_P0)
  [VehConfig] -> Cruise/4(VehConfig)
  [Target_Line] -> Cruise/12(Target_Line)
  [HWAStateInfo] -> Unit Delay2/1
  [AD_CAN] -> ESS/3(AD_CAN)
  Cruise/1(EDR_Longitude_HWAExit) -> [EDR_Longitude_HWAExit]
  [VehicleSts] -> ESS/2(VehicleSts)
  [ELK_Obj] -> LSS/10(ELK_Obj)
  [Fusion_Line] -> LSS/7(Fusion_Line)
  [HWAStateInfo] -> Unit Delay3/1
  [AEB_OBJ] -> ESS/5(AEB_OBJ)
  [LatStateInfo] -> Unit Delay4/1
  [AD_CAN] -> HOD/1(EPS_DrvInpTrqVal_HighReslolution)
  [BusLatCtrlInfo] -> LSS/11(BusLatCtrlInfo)
  [DriverSts] -> Cruise/7(DriverSts)
  PLAN_DPC_ESS/1 -> ESS/1(ESS_SideViewSts)
  w2/1 -> SetSpeedKmh/1  "SetSpeedKmh"
  Cruise/2(UOMSysFeedBack) -> [UOMSysFeedBack]
  [UOMSysFeedBack] -> Unit Delay/1
  [AD_CAN] -> UOM/1(CSA)
  UOM/1(UserOperation) -> [UserOperation], Cruise/3(UserOperation)
  Bus Selector24/2 -> w461/1  "<VSM_HWA_LaneChangeReq>"
  [UserOperation] -> Bus Selector5/1
  Unit Delay/1 -> UOM/2(FunFeedBack)
  Direct Lookup Table (n-D)/1 -> Switch5/3
  [ESSState] -> Cruise/13(ESSState)
  Bus Selector19/20 -> w3/1  "<Signal_HWATextDisp>"
  PilotSts/1 -> [PilotSts]
  [PilotSts] -> Cruise/14(PilotSts)
  Constant/1 -> OR/1
  LKASwtReq/1 -> OR/2  "LKASwtReq"
  LCKSwtReq/1 -> OR1/2  "LCKSwtReq"
  Constant2/1 -> OR1/1
  ELKSwtReq/1 -> OR2/2  "ELKSwtReq"
  Constant3/1 -> OR2/1
  ESS_PedSwtReq/1 -> Bus Creator3/96  "ESS_PedSwtReq"
  ESS_VehSwtReq/1 -> OR4/2  "ESS_VehSwtReq"
  LDWSwtReq/1 -> OR5/2  "LDWSwtReq"
  TSRSwtReq/1 -> OR6/2  "TSRSwtReq"
  TSRWarnSwtReq/1 -> OR7/2  "TSRWarnSwtReq"
  ICA_HandsOffSwtReq/1 -> OR8/2  "ICA_HandsOffSwtReq"
  ISLSwtReq/1 -> OR9/2  "ISLSwtReq"
  TSR_SnvtySet/1 -> Bus Creator3/103  "TSR_SnvtySet"
  LSSWarnFormSwtReq/1 -> Bus Creator3/104  "LSSWarnFormSwtReq"
  LSSSwtReq/1 -> OR14/2  "LSSSwtReq"
  IntelligentEvaSwtReq/1 -> OR15/2  "IntelligentEvaSwtReq"
  AESSwtReq/1 -> OR12/2  "AESSwtReq"
  HWA_SnvtySet/1 -> Bus Creator3/109  "HWA_SnvtySet"
  Constant5/1 -> OR4/1
  Constant6/1 -> OR5/1
  Constant7/1 -> OR6/1
  Constant8/1 -> OR7/1
  Constant9/1 -> OR8/1
  Constant10/1 -> OR9/1
  Constant12/1 -> OR14/1
  Constant13/1 -> OR15/1
  Constant14/1 -> OR12/1
  [DirverOverride] -> Bus Assignment/10, Compare To Zero/1
